simulink model "model"  (R2014a)
(part 7 of 8)

      | %<ID>
      | %<Vbase>V
      | %<VLF>pu
      | %<angleLF>deg.
      | %<Name>
  bus357 : powerlib/Measurements/Load Flow Bus  LConnTagsString=a  ID=bus357  Vbase=110000  Vref=1  Vangle=0  VLF=1  angleLF=0
      settings: AttributesFormatString=|
      | %<ID>
      | %<Vbase>V
      | %<VLF>pu
      | %<angleLF>deg.
      | %<Name>
  bus358 : powerlib/Measurements/Load Flow Bus  LConnTagsString=a  ID=bus358  Vbase=110000  Vref=1  Vangle=0  VLF=1  angleLF=0
      settings: AttributesFormatString=|
      | %<ID>
      | %<Vbase>V
      | %<VLF>pu
      | %<angleLF>deg.
      | %<Name>
  bus359 : powerlib/Measurements/Load Flow Bus  LConnTagsString=a  ID=bus359  Vbase=110000  Vref=1  Vangle=0  VLF=1  angleLF=0
      settings: AttributesFormatString=|
      | %<ID>
      | %<Vbase>V
      | %<VLF>pu
      | %<angleLF>deg.
      | %<Name>
  bus36 : powerlib/Measurements/Load Flow Bus  LConnTagsString=a  ID=bus36  Vbase=110000  Vref=1  Vangle=0  VLF=1  angleLF=0
      settings: AttributesFormatString=|
      | %<ID>
      | %<Vbase>V
      | %<VLF>pu
      | %<angleLF>deg.
      | %<Name>
  bus360 : powerlib/Measurements/Load Flow Bus  LConnTagsString=a  ID=bus360  Vbase=110000  Vref=1  Vangle=0  VLF=1  angleLF=0
      settings: AttributesFormatString=|
      | %<ID>
      | %<Vbase>V
      | %<VLF>pu
      | %<angleLF>deg.
      | %<Name>
  bus361 : powerlib/Measurements/Load Flow Bus  LConnTagsString=a  ID=bus361  Vbase=110000  Vref=1  Vangle=0  VLF=1  angleLF=0
      settings: AttributesFormatString=|
      | %<ID>
      | %<Vbase>V
      | %<VLF>pu
      | %<angleLF>deg.
      | %<Name>
  bus362 : powerlib/Measurements/Load Flow Bus  LConnTagsString=a  ID=bus362  Vbase=110000  Vref=1  Vangle=0  VLF=1  angleLF=0
      settings: AttributesFormatString=|
      | %<ID>
      | %<Vbase>V
      | %<VLF>pu
      | %<angleLF>deg.
      | %<Name>
  bus363 : powerlib/Measurements/Load Flow Bus  LConnTagsString=a  ID=bus363  Vbase=110000  Vref=1  Vangle=0  VLF=1  angleLF=0
      settings: AttributesFormatString=|
      | %<ID>
      | %<Vbase>V
      | %<VLF>pu
      | %<angleLF>deg.
      | %<Name>
  bus364 : powerlib/Measurements/Load Flow Bus  LConnTagsString=a  ID=bus364  Vbase=110000  Vref=1  Vangle=0  VLF=1  angleLF=0
      settings: AttributesFormatString=|
      | %<ID>
      | %<Vbase>V
      | %<VLF>pu
      | %<angleLF>deg.
      | %<Name>
  bus365 : powerlib/Measurements/Load Flow Bus  LConnTagsString=a  ID=bus365  Vbase=110000  Vref=1  Vangle=0  VLF=1  angleLF=0
      settings: AttributesFormatString=|
      | %<ID>
      | %<Vbase>V
      | %<VLF>pu
      | %<angleLF>deg.
      | %<Name>
  bus366 : powerlib/Measurements/Load Flow Bus  LConnTagsString=a  ID=bus366  Vbase=110000  Vref=1  Vangle=0  VLF=1  angleLF=0
      settings: AttributesFormatString=|
      | %<ID>
      | %<Vbase>V
      | %<VLF>pu
      | %<angleLF>deg.
      | %<Name>
  bus367 : powerlib/Measurements/Load Flow Bus  LConnTagsString=a  ID=bus367  Vbase=110000  Vref=1  Vangle=0  VLF=1  angleLF=0
      settings: AttributesFormatString=|
      | %<ID>
      | %<Vbase>V
      | %<VLF>pu
      | %<angleLF>deg.
      | %<Name>
  bus368 : powerlib/Measurements/Load Flow Bus  LConnTagsString=a  ID=bus368  Vbase=110000  Vref=1  Vangle=0  VLF=1  angleLF=0
      settings: AttributesFormatString=|
      | %<ID>
      | %<Vbase>V
      | %<VLF>pu
      | %<angleLF>deg.
      | %<Name>
  bus369 : powerlib/Measurements/Load Flow Bus  LConnTagsString=a  ID=bus369  Vbase=110000  Vref=1  Vangle=0  VLF=1  angleLF=0
      settings: AttributesFormatString=|
      | %<ID>
      | %<Vbase>V
      | %<VLF>pu
      | %<angleLF>deg.
      | %<Name>
  bus37 : powerlib/Measurements/Load Flow Bus  LConnTagsString=a  ID=bus37  Vbase=110000  Vref=1  Vangle=0  VLF=1  angleLF=0
      settings: AttributesFormatString=|
      | %<ID>
      | %<Vbase>V
      | %<VLF>pu
      | %<angleLF>deg.
      | %<Name>
  bus370 : powerlib/Measurements/Load Flow Bus  LConnTagsString=a  ID=bus370  Vbase=110000  Vref=1  Vangle=0  VLF=1  angleLF=0
      settings: AttributesFormatString=|
      | %<ID>
      | %<Vbase>V
      | %<VLF>pu
      | %<angleLF>deg.
      | %<Name>
  bus371 : powerlib/Measurements/Load Flow Bus  LConnTagsString=a  ID=bus371  Vbase=110000  Vref=1  Vangle=0  VLF=1  angleLF=0
      settings: AttributesFormatString=|
      | %<ID>
      | %<Vbase>V
      | %<VLF>pu
      | %<angleLF>deg.
      | %<Name>
  bus372 : powerlib/Measurements/Load Flow Bus  LConnTagsString=a  ID=bus372  Vbase=110000  Vref=1  Vangle=0  VLF=1  angleLF=0
      settings: AttributesFormatString=|
      | %<ID>
      | %<Vbase>V
      | %<VLF>pu
      | %<angleLF>deg.
      | %<Name>
  bus373 : powerlib/Measurements/Load Flow Bus  LConnTagsString=a  ID=bus373  Vbase=110000  Vref=1  Vangle=0  VLF=1  angleLF=0
      settings: AttributesFormatString=|
      | %<ID>
      | %<Vbase>V
      | %<VLF>pu
      | %<angleLF>deg.
      | %<Name>
  bus374 : powerlib/Measurements/Load Flow Bus  LConnTagsString=a  ID=bus374  Vbase=110000  Vref=1  Vangle=0  VLF=1  angleLF=0
      settings: AttributesFormatString=|
      | %<ID>
      | %<Vbase>V
      | %<VLF>pu
      | %<angleLF>deg.
      | %<Name>
  bus375 : powerlib/Measurements/Load Flow Bus  LConnTagsString=a  ID=bus375  Vbase=110000  Vref=1  Vangle=0  VLF=1  angleLF=0
      settings: AttributesFormatString=|
      | %<ID>
      | %<Vbase>V
      | %<VLF>pu
      | %<angleLF>deg.
      | %<Name>
  bus376 : powerlib/Measurements/Load Flow Bus  LConnTagsString=a  ID=bus376  Vbase=110000  Vref=1  Vangle=0  VLF=1  angleLF=0
      settings: AttributesFormatString=|
      | %<ID>
      | %<Vbase>V
      | %<VLF>pu
      | %<angleLF>deg.
      | %<Name>
  bus377 : powerlib/Measurements/Load Flow Bus  LConnTagsString=a  ID=bus377  Vbase=110000  Vref=1  Vangle=0  VLF=1  angleLF=0
      settings: AttributesFormatString=|
      | %<ID>
      | %<Vbase>V
      | %<VLF>pu
      | %<angleLF>deg.
      | %<Name>
  bus378 : powerlib/Measurements/Load Flow Bus  LConnTagsString=a  ID=bus378  Vbase=110000  Vref=1  Vangle=0  VLF=1  angleLF=0
      settings: AttributesFormatString=|
      | %<ID>
      | %<Vbase>V
      | %<VLF>pu
      | %<angleLF>deg.
      | %<Name>
  bus379 : powerlib/Measurements/Load Flow Bus  LConnTagsString=a  ID=bus379  Vbase=110000  Vref=1  Vangle=0  VLF=1  angleLF=0
      settings: AttributesFormatString=|
      | %<ID>
      | %<Vbase>V
      | %<VLF>pu
      | %<angleLF>deg.
      | %<Name>
  bus38 : powerlib/Measurements/Load Flow Bus  LConnTagsString=a  ID=bus38  Vbase=110000  Vref=1  Vangle=0  VLF=1  angleLF=0
      settings: AttributesFormatString=|
      | %<ID>
      | %<Vbase>V
      | %<VLF>pu
      | %<angleLF>deg.
      | %<Name>
  bus380 : powerlib/Measurements/Load Flow Bus  LConnTagsString=a  ID=bus380  Vbase=110000  Vref=1  Vangle=0  VLF=1  angleLF=0
      settings: AttributesFormatString=|
      | %<ID>
      | %<Vbase>V
      | %<VLF>pu
      | %<angleLF>deg.
      | %<Name>
  bus381 : powerlib/Measurements/Load Flow Bus  LConnTagsString=a  ID=bus381  Vbase=110000  Vref=1  Vangle=0  VLF=1  angleLF=0
      settings: AttributesFormatString=|
      | %<ID>
      | %<Vbase>V
      | %<VLF>pu
      | %<angleLF>deg.
      | %<Name>
  bus382 : powerlib/Measurements/Load Flow Bus  LConnTagsString=a  ID=bus382  Vbase=110000  Vref=1  Vangle=0  VLF=1  angleLF=0
      settings: AttributesFormatString=|
      | %<ID>
      | %<Vbase>V
      | %<VLF>pu
      | %<angleLF>deg.
      | %<Name>
  bus383 : powerlib/Measurements/Load Flow Bus  LConnTagsString=a  ID=bus383  Vbase=110000  Vref=1  Vangle=0  VLF=1  angleLF=0
      settings: AttributesFormatString=|
      | %<ID>
      | %<Vbase>V
      | %<VLF>pu
      | %<angleLF>deg.
      | %<Name>
  bus384 : powerlib/Measurements/Load Flow Bus  LConnTagsString=a  ID=bus384  Vbase=110000  Vref=1  Vangle=0  VLF=1  angleLF=0
      settings: AttributesFormatString=|
      | %<ID>
      | %<Vbase>V
      | %<VLF>pu
      | %<angleLF>deg.
      | %<Name>
  bus385 : powerlib/Measurements/Load Flow Bus  LConnTagsString=a  ID=bus385  Vbase=110000  Vref=1  Vangle=0  VLF=1  angleLF=0
      settings: AttributesFormatString=|
      | %<ID>
      | %<Vbase>V
      | %<VLF>pu
      | %<angleLF>deg.
      | %<Name>
  bus386 : powerlib/Measurements/Load Flow Bus  LConnTagsString=a  ID=bus386  Vbase=110000  Vref=1  Vangle=0  VLF=1  angleLF=0
      settings: AttributesFormatString=|
      | %<ID>
      | %<Vbase>V
      | %<VLF>pu
      | %<angleLF>deg.
      | %<Name>
  bus387 : powerlib/Measurements/Load Flow Bus  LConnTagsString=a  ID=bus387  Vbase=110000  Vref=1  Vangle=0  VLF=1  angleLF=0
      settings: AttributesFormatString=|
      | %<ID>
      | %<Vbase>V
      | %<VLF>pu
      | %<angleLF>deg.
      | %<Name>
  bus388 : powerlib/Measurements/Load Flow Bus  LConnTagsString=a  ID=bus388  Vbase=110000  Vref=1  Vangle=0  VLF=1  angleLF=0
      settings: AttributesFormatString=|
      | %<ID>
      | %<Vbase>V
      | %<VLF>pu
      | %<angleLF>deg.
      | %<Name>
  bus389 : powerlib/Measurements/Load Flow Bus  LConnTagsString=a  ID=bus389  Vbase=110000  Vref=1  Vangle=0  VLF=1  angleLF=0
      settings: AttributesFormatString=|
      | %<ID>
      | %<Vbase>V
      | %<VLF>pu
      | %<angleLF>deg.
      | %<Name>
  bus39 : powerlib/Measurements/Load Flow Bus  LConnTagsString=a  ID=bus39  Vbase=110000  Vref=1  Vangle=0  VLF=1  angleLF=0
      settings: AttributesFormatString=|
      | %<ID>
      | %<Vbase>V
      | %<VLF>pu
      | %<angleLF>deg.
      | %<Name>
  bus390 : powerlib/Measurements/Load Flow Bus  LConnTagsString=a  ID=bus390  Vbase=110000  Vref=1  Vangle=0  VLF=1  angleLF=0
      settings: AttributesFormatString=|
      | %<ID>
      | %<Vbase>V
      | %<VLF>pu
      | %<angleLF>deg.
      | %<Name>
  bus391 : powerlib/Measurements/Load Flow Bus  LConnTagsString=a  ID=bus391  Vbase=110000  Vref=1  Vangle=0  VLF=1  angleLF=0
      settings: AttributesFormatString=|
      | %<ID>
      | %<Vbase>V
      | %<VLF>pu
      | %<angleLF>deg.
      | %<Name>
  bus392 : powerlib/Measurements/Load Flow Bus  LConnTagsString=a  ID=bus392  Vbase=110000  Vref=1  Vangle=0  VLF=1  angleLF=0
      settings: AttributesFormatString=|
      | %<ID>
      | %<Vbase>V
      | %<VLF>pu
      | %<angleLF>deg.
      | %<Name>
  bus393 : powerlib/Measurements/Load Flow Bus  LConnTagsString=a  ID=bus393  Vbase=110000  Vref=1  Vangle=0  VLF=1  angleLF=0
      settings: AttributesFormatString=|
      | %<ID>
      | %<Vbase>V
      | %<VLF>pu
      | %<angleLF>deg.
      | %<Name>
  bus394 : powerlib/Measurements/Load Flow Bus  LConnTagsString=a  ID=bus394  Vbase=110000  Vref=1  Vangle=0  VLF=1  angleLF=0
      settings: AttributesFormatString=|
      | %<ID>
      | %<Vbase>V
      | %<VLF>pu
      | %<angleLF>deg.
      | %<Name>
  bus395 : powerlib/Measurements/Load Flow Bus  LConnTagsString=a  ID=bus395  Vbase=110000  Vref=1  Vangle=0  VLF=1  angleLF=0
      settings: AttributesFormatString=|
      | %<ID>
      | %<Vbase>V
      | %<VLF>pu
      | %<angleLF>deg.
      | %<Name>
  bus396 : powerlib/Measurements/Load Flow Bus  LConnTagsString=a  ID=bus396  Vbase=110000  Vref=1  Vangle=0  VLF=1  angleLF=0
      settings: AttributesFormatString=|
      | %<ID>
      | %<Vbase>V
      | %<VLF>pu
      | %<angleLF>deg.
      | %<Name>
  bus397 : powerlib/Measurements/Load Flow Bus  LConnTagsString=a  ID=bus397  Vbase=110000  Vref=1  Vangle=0  VLF=1  angleLF=0
      settings: AttributesFormatString=|
      | %<ID>
      | %<Vbase>V
      | %<VLF>pu
      | %<angleLF>deg.
      | %<Name>
  bus398 : powerlib/Measurements/Load Flow Bus  LConnTagsString=a  ID=bus398  Vbase=110000  Vref=1  Vangle=0  VLF=1  angleLF=0
      settings: AttributesFormatString=|
      | %<ID>
      | %<Vbase>V
      | %<VLF>pu
      | %<angleLF>deg.
      | %<Name>
  bus399 : powerlib/Measurements/Load Flow Bus  LConnTagsString=a  ID=bus399  Vbase=110000  Vref=1  Vangle=0  VLF=1  angleLF=0
      settings: AttributesFormatString=|
      | %<ID>
      | %<Vbase>V
      | %<VLF>pu
      | %<angleLF>deg.
      | %<Name>
  bus4 : powerlib/Measurements/Load Flow Bus  LConnTagsString=a  ID=bus4  Vbase=20000  Vref=1  Vangle=0  VLF=1  angleLF=0
      settings: AttributesFormatString=|
      | %<ID>
      | %<Vbase>V
      | %<VLF>pu
      | %<angleLF>deg.
      | %<Name>
  bus40 : powerlib/Measurements/Load Flow Bus  LConnTagsString=a  ID=bus40  Vbase=110000  Vref=1  Vangle=0  VLF=1  angleLF=0
      settings: AttributesFormatString=|
      | %<ID>
      | %<Vbase>V
      | %<VLF>pu
      | %<angleLF>deg.
      | %<Name>
  bus400 : powerlib/Measurements/Load Flow Bus  LConnTagsString=a  ID=bus400  Vbase=110000  Vref=1  Vangle=0  VLF=1  angleLF=0
      settings: AttributesFormatString=|
      | %<ID>
      | %<Vbase>V
      | %<VLF>pu
      | %<angleLF>deg.
      | %<Name>
  bus401 : powerlib/Measurements/Load Flow Bus  LConnTagsString=a  ID=bus401  Vbase=110000  Vref=1  Vangle=0  VLF=1  angleLF=0
      settings: AttributesFormatString=|
      | %<ID>
      | %<Vbase>V
      | %<VLF>pu
      | %<angleLF>deg.
      | %<Name>
  bus402 : powerlib/Measurements/Load Flow Bus  LConnTagsString=a  ID=bus402  Vbase=110000  Vref=1  Vangle=0  VLF=1  angleLF=0
      settings: AttributesFormatString=|
      | %<ID>
      | %<Vbase>V
      | %<VLF>pu
      | %<angleLF>deg.
      | %<Name>
  bus403 : powerlib/Measurements/Load Flow Bus  LConnTagsString=a  ID=bus403  Vbase=110000  Vref=1  Vangle=0  VLF=1  angleLF=0
      settings: AttributesFormatString=|
      | %<ID>
      | %<Vbase>V
      | %<VLF>pu
      | %<angleLF>deg.
      | %<Name>
  bus404 : powerlib/Measurements/Load Flow Bus  LConnTagsString=a  ID=bus404  Vbase=110000  Vref=1  Vangle=0  VLF=1  angleLF=0
      settings: AttributesFormatString=|
      | %<ID>
      | %<Vbase>V
      | %<VLF>pu
      | %<angleLF>deg.
      | %<Name>
  bus405 : powerlib/Measurements/Load Flow Bus  LConnTagsString=a  ID=bus405  Vbase=110000  Vref=1  Vangle=0  VLF=1  angleLF=0
      settings: AttributesFormatString=|
      | %<ID>
      | %<Vbase>V
      | %<VLF>pu
      | %<angleLF>deg.
      | %<Name>
  bus406 : powerlib/Measurements/Load Flow Bus  LConnTagsString=a  ID=bus406  Vbase=110000  Vref=1  Vangle=0  VLF=1  angleLF=0
      settings: AttributesFormatString=|
      | %<ID>
      | %<Vbase>V
      | %<VLF>pu
      | %<angleLF>deg.
      | %<Name>
  bus407 : powerlib/Measurements/Load Flow Bus  LConnTagsString=a  ID=bus407  Vbase=110000  Vref=1  Vangle=0  VLF=1  angleLF=0
      settings: AttributesFormatString=|
      | %<ID>
      | %<Vbase>V
      | %<VLF>pu
      | %<angleLF>deg.
      | %<Name>
  bus408 : powerlib/Measurements/Load Flow Bus  LConnTagsString=a  ID=bus408  Vbase=110000  Vref=1  Vangle=0  VLF=1  angleLF=0
      settings: AttributesFormatString=|
      | %<ID>
      | %<Vbase>V
      | %<VLF>pu
      | %<angleLF>deg.
      | %<Name>
  bus409 : powerlib/Measurements/Load Flow Bus  LConnTagsString=a  ID=bus409  Vbase=110000  Vref=1  Vangle=0  VLF=1  angleLF=0
      settings: AttributesFormatString=|
      | %<ID>
      | %<Vbase>V
      | %<VLF>pu
      | %<angleLF>deg.
      | %<Name>
  bus41 : powerlib/Measurements/Load Flow Bus  LConnTagsString=a  ID=bus41  Vbase=110000  Vref=1  Vangle=0  VLF=1  angleLF=0
      settings: AttributesFormatString=|
      | %<ID>
      | %<Vbase>V
      | %<VLF>pu
      | %<angleLF>deg.
      | %<Name>
  bus410 : powerlib/Measurements/Load Flow Bus  LConnTagsString=a  ID=bus410  Vbase=110000  Vref=1  Vangle=0  VLF=1  angleLF=0
      settings: AttributesFormatString=|
      | %<ID>
      | %<Vbase>V
      | %<VLF>pu
      | %<angleLF>deg.
      | %<Name>
  bus411 : powerlib/Measurements/Load Flow Bus  LConnTagsString=a  ID=bus411  Vbase=110000  Vref=1  Vangle=0  VLF=1  angleLF=0
      settings: AttributesFormatString=|
      | %<ID>
      | %<Vbase>V
      | %<VLF>pu
      | %<angleLF>deg.
      | %<Name>
  bus412 : powerlib/Measurements/Load Flow Bus  LConnTagsString=a  ID=bus412  Vbase=110000  Vref=1  Vangle=0  VLF=1  angleLF=0
      settings: AttributesFormatString=|
      | %<ID>
      | %<Vbase>V
      | %<VLF>pu
      | %<angleLF>deg.
      | %<Name>
  bus413 : powerlib/Measurements/Load Flow Bus  LConnTagsString=a  ID=bus413  Vbase=110000  Vref=1  Vangle=0  VLF=1  angleLF=0
      settings: AttributesFormatString=|
      | %<ID>
      | %<Vbase>V
      | %<VLF>pu
      | %<angleLF>deg.
      | %<Name>
  bus414 : powerlib/Measurements/Load Flow Bus  LConnTagsString=a  ID=bus414  Vbase=110000  Vref=1  Vangle=0  VLF=1  angleLF=0
      settings: AttributesFormatString=|
      | %<ID>
      | %<Vbase>V
      | %<VLF>pu
      | %<angleLF>deg.
      | %<Name>
  bus415 : powerlib/Measurements/Load Flow Bus  LConnTagsString=a  ID=bus415  Vbase=110000  Vref=1  Vangle=0  VLF=1  angleLF=0
      settings: AttributesFormatString=|
      | %<ID>
      | %<Vbase>V
      | %<VLF>pu
      | %<angleLF>deg.
      | %<Name>
  bus416 : powerlib/Measurements/Load Flow Bus  LConnTagsString=a  ID=bus416  Vbase=110000  Vref=1  Vangle=0  VLF=1  angleLF=0
      settings: AttributesFormatString=|
      | %<ID>
      | %<Vbase>V
      | %<VLF>pu
      | %<angleLF>deg.
      | %<Name>
  bus417 : powerlib/Measurements/Load Flow Bus  LConnTagsString=a  ID=bus417  Vbase=110000  Vref=1  Vangle=0  VLF=1  angleLF=0
      settings: AttributesFormatString=|
      | %<ID>
      | %<Vbase>V
      | %<VLF>pu
      | %<angleLF>deg.
      | %<Name>
  bus418 : powerlib/Measurements/Load Flow Bus  LConnTagsString=a  ID=bus418  Vbase=110000  Vref=1  Vangle=0  VLF=1  angleLF=0
      settings: AttributesFormatString=|
      | %<ID>
      | %<Vbase>V
      | %<VLF>pu
      | %<angleLF>deg.
      | %<Name>
  bus419 : powerlib/Measurements/Load Flow Bus  LConnTagsString=a  ID=bus419  Vbase=110000  Vref=1  Vangle=0  VLF=1  angleLF=0
      settings: AttributesFormatString=|
      | %<ID>
      | %<Vbase>V
      | %<VLF>pu
      | %<angleLF>deg.
      | %<Name>
  bus42 : powerlib/Measurements/Load Flow Bus  LConnTagsString=a  ID=bus42  Vbase=110000  Vref=1  Vangle=0  VLF=1  angleLF=0
      settings: AttributesFormatString=|
      | %<ID>
      | %<Vbase>V
      | %<VLF>pu
      | %<angleLF>deg.
      | %<Name>
  bus420 : powerlib/Measurements/Load Flow Bus  LConnTagsString=a  ID=bus420  Vbase=110000  Vref=1  Vangle=0  VLF=1  angleLF=0
      settings: AttributesFormatString=|
      | %<ID>
      | %<Vbase>V
      | %<VLF>pu
      | %<angleLF>deg.
      | %<Name>
  bus421 : powerlib/Measurements/Load Flow Bus  LConnTagsString=a  ID=bus421  Vbase=110000  Vref=1  Vangle=0  VLF=1  angleLF=0
      settings: AttributesFormatString=|
      | %<ID>
      | %<Vbase>V
      | %<VLF>pu
      | %<angleLF>deg.
      | %<Name>
  bus422 : powerlib/Measurements/Load Flow Bus  LConnTagsString=a  ID=bus422  Vbase=110000  Vref=1  Vangle=0  VLF=1  angleLF=0
      settings: AttributesFormatString=|
      | %<ID>
      | %<Vbase>V
      | %<VLF>pu
      | %<angleLF>deg.
      | %<Name>
  bus423 : powerlib/Measurements/Load Flow Bus  LConnTagsString=a  ID=bus423  Vbase=110000  Vref=1  Vangle=0  VLF=1  angleLF=0
      settings: AttributesFormatString=|
      | %<ID>
      | %<Vbase>V
      | %<VLF>pu
      | %<angleLF>deg.
      | %<Name>
  bus424 : powerlib/Measurements/Load Flow Bus  LConnTagsString=a  ID=bus424  Vbase=110000  Vref=1  Vangle=0  VLF=1  angleLF=0
      settings: AttributesFormatString=|
      | %<ID>
      | %<Vbase>V
      | %<VLF>pu
      | %<angleLF>deg.
      | %<Name>
  bus425 : powerlib/Measurements/Load Flow Bus  LConnTagsString=a  ID=bus425  Vbase=110000  Vref=1  Vangle=0  VLF=1  angleLF=0
      settings: AttributesFormatString=|
      | %<ID>
      | %<Vbase>V
      | %<VLF>pu
      | %<angleLF>deg.
      | %<Name>
  bus426 : powerlib/Measurements/Load Flow Bus  LConnTagsString=a  ID=bus426  Vbase=110000  Vref=1  Vangle=0  VLF=1  angleLF=0
      settings: AttributesFormatString=|
      | %<ID>
      | %<Vbase>V
      | %<VLF>pu
      | %<angleLF>deg.
      | %<Name>
  bus427 : powerlib/Measurements/Load Flow Bus  LConnTagsString=a  ID=bus427  Vbase=110000  Vref=1  Vangle=0  VLF=1  angleLF=0
      settings: AttributesFormatString=|
      | %<ID>
      | %<Vbase>V
      | %<VLF>pu
      | %<angleLF>deg.
      | %<Name>
  bus428 : powerlib/Measurements/Load Flow Bus  LConnTagsString=a  ID=bus428  Vbase=110000  Vref=1  Vangle=0  VLF=1  angleLF=0
      settings: AttributesFormatString=|
      | %<ID>
      | %<Vbase>V
      | %<VLF>pu
      | %<angleLF>deg.
      | %<Name>
  bus429 : powerlib/Measurements/Load Flow Bus  LConnTagsString=a  ID=bus429  Vbase=110000  Vref=1  Vangle=0  VLF=1  angleLF=0
      settings: AttributesFormatString=|
      | %<ID>
      | %<Vbase>V
      | %<VLF>pu
      | %<angleLF>deg.
      | %<Name>
  bus43 : powerlib/Measurements/Load Flow Bus  LConnTagsString=a  ID=bus43  Vbase=110000  Vref=1  Vangle=0  VLF=1  angleLF=0
      settings: AttributesFormatString=|
      | %<ID>
      | %<Vbase>V
      | %<VLF>pu
      | %<angleLF>deg.
      | %<Name>
  bus430 : powerlib/Measurements/Load Flow Bus  LConnTagsString=a  ID=bus430  Vbase=110000  Vref=1  Vangle=0  VLF=1  angleLF=0
      settings: AttributesFormatString=|
      | %<ID>
      | %<Vbase>V
      | %<VLF>pu
      | %<angleLF>deg.
      | %<Name>
  bus431 : powerlib/Measurements/Load Flow Bus  LConnTagsString=a  ID=bus431  Vbase=110000  Vref=1  Vangle=0  VLF=1  angleLF=0
      settings: AttributesFormatString=|
      | %<ID>
      | %<Vbase>V
      | %<VLF>pu
      | %<angleLF>deg.
      | %<Name>
  bus432 : powerlib/Measurements/Load Flow Bus  LConnTagsString=a  ID=bus432  Vbase=110000  Vref=1  Vangle=0  VLF=1  angleLF=0
      settings: AttributesFormatString=|
      | %<ID>
      | %<Vbase>V
      | %<VLF>pu
      | %<angleLF>deg.
      | %<Name>
  bus433 : powerlib/Measurements/Load Flow Bus  LConnTagsString=a  ID=bus433  Vbase=110000  Vref=1  Vangle=0  VLF=1  angleLF=0
      settings: AttributesFormatString=|
      | %<ID>
      | %<Vbase>V
      | %<VLF>pu
      | %<angleLF>deg.
      | %<Name>
  bus434 : powerlib/Measurements/Load Flow Bus  LConnTagsString=a  ID=bus434  Vbase=110000  Vref=1  Vangle=0  VLF=1  angleLF=0
      settings: AttributesFormatString=|
      | %<ID>
      | %<Vbase>V
      | %<VLF>pu
      | %<angleLF>deg.
      | %<Name>
  bus435 : powerlib/Measurements/Load Flow Bus  LConnTagsString=a  ID=bus435  Vbase=110000  Vref=1  Vangle=0  VLF=1  angleLF=0
      settings: AttributesFormatString=|
      | %<ID>
      | %<Vbase>V
      | %<VLF>pu
      | %<angleLF>deg.
      | %<Name>
  bus436 : powerlib/Measurements/Load Flow Bus  LConnTagsString=a  ID=bus436  Vbase=110000  Vref=1  Vangle=0  VLF=1  angleLF=0
      settings: AttributesFormatString=|
      | %<ID>
      | %<Vbase>V
      | %<VLF>pu
      | %<angleLF>deg.
      | %<Name>
  bus437 : powerlib/Measurements/Load Flow Bus  LConnTagsString=a  ID=bus437  Vbase=110000  Vref=1  Vangle=0  VLF=1  angleLF=0
      settings: AttributesFormatString=|
      | %<ID>
      | %<Vbase>V
      | %<VLF>pu
      | %<angleLF>deg.
      | %<Name>
  bus438 : powerlib/Measurements/Load Flow Bus  LConnTagsString=a  ID=bus438  Vbase=110000  Vref=1  Vangle=0  VLF=1  angleLF=0
      settings: AttributesFormatString=|
      | %<ID>
      | %<Vbase>V
      | %<VLF>pu
      | %<angleLF>deg.
      | %<Name>
  bus439 : powerlib/Measurements/Load Flow Bus  LConnTagsString=a  ID=bus439  Vbase=110000  Vref=1  Vangle=0  VLF=1  angleLF=0
      settings: AttributesFormatString=|
      | %<ID>
      | %<Vbase>V
      | %<VLF>pu
      | %<angleLF>deg.
      | %<Name>
  bus44 : powerlib/Measurements/Load Flow Bus  LConnTagsString=a  ID=bus44  Vbase=110000  Vref=1  Vangle=0  VLF=1  angleLF=0
      settings: AttributesFormatString=|
      | %<ID>
      | %<Vbase>V
      | %<VLF>pu
      | %<angleLF>deg.
      | %<Name>
  bus440 : powerlib/Measurements/Load Flow Bus  LConnTagsString=a  ID=bus440  Vbase=110000  Vref=1  Vangle=0  VLF=1  angleLF=0
      settings: AttributesFormatString=|
      | %<ID>
      | %<Vbase>V
      | %<VLF>pu
      | %<angleLF>deg.
      | %<Name>
  bus441 : powerlib/Measurements/Load Flow Bus  LConnTagsString=a  ID=bus441  Vbase=110000  Vref=1  Vangle=0  VLF=1  angleLF=0
      settings: AttributesFormatString=|
      | %<ID>
      | %<Vbase>V
      | %<VLF>pu
      | %<angleLF>deg.
      | %<Name>
  bus442 : powerlib/Measurements/Load Flow Bus  LConnTagsString=a  ID=bus442  Vbase=110000  Vref=1  Vangle=0  VLF=1  angleLF=0
      settings: AttributesFormatString=|
      | %<ID>
      | %<Vbase>V
      | %<VLF>pu
      | %<angleLF>deg.
      | %<Name>
  bus443 : powerlib/Measurements/Load Flow Bus  LConnTagsString=a  ID=bus443  Vbase=110000  Vref=1  Vangle=0  VLF=1  angleLF=0
      settings: AttributesFormatString=|
      | %<ID>
      | %<Vbase>V
      | %<VLF>pu
      | %<angleLF>deg.
      | %<Name>
  bus444 : powerlib/Measurements/Load Flow Bus  LConnTagsString=a  ID=bus444  Vbase=110000  Vref=1  Vangle=0  VLF=1  angleLF=0
      settings: AttributesFormatString=|
      | %<ID>
      | %<Vbase>V
      | %<VLF>pu
      | %<angleLF>deg.
      | %<Name>
  bus445 : powerlib/Measurements/Load Flow Bus  LConnTagsString=a  ID=bus445  Vbase=110000  Vref=1  Vangle=0  VLF=1  angleLF=0
      settings: AttributesFormatString=|
      | %<ID>
      | %<Vbase>V
      | %<VLF>pu
      | %<angleLF>deg.
      | %<Name>
  bus446 : powerlib/Measurements/Load Flow Bus  LConnTagsString=a  ID=bus446  Vbase=110000  Vref=1  Vangle=0  VLF=1  angleLF=0
      settings: AttributesFormatString=|
      | %<ID>
      | %<Vbase>V
      | %<VLF>pu
      | %<angleLF>deg.
      | %<Name>
  bus447 : powerlib/Measurements/Load Flow Bus  LConnTagsString=a  ID=bus447  Vbase=110000  Vref=1  Vangle=0  VLF=1  angleLF=0
      settings: AttributesFormatString=|
      | %<ID>
      | %<Vbase>V
      | %<VLF>pu
      | %<angleLF>deg.
      | %<Name>
  bus448 : powerlib/Measurements/Load Flow Bus  LConnTagsString=a  ID=bus448  Vbase=110000  Vref=1  Vangle=0  VLF=1  angleLF=0
      settings: AttributesFormatString=|
      | %<ID>
      | %<Vbase>V
      | %<VLF>pu
      | %<angleLF>deg.
      | %<Name>
  bus449 : powerlib/Measurements/Load Flow Bus  LConnTagsString=a  ID=bus449  Vbase=110000  Vref=1  Vangle=0  VLF=1  angleLF=0
      settings: AttributesFormatString=|
      | %<ID>
      | %<Vbase>V
      | %<VLF>pu
      | %<angleLF>deg.
      | %<Name>
  bus45 : powerlib/Measurements/Load Flow Bus  LConnTagsString=a  ID=bus45  Vbase=110000  Vref=1  Vangle=0  VLF=1  angleLF=0
      settings: AttributesFormatString=|
      | %<ID>
      | %<Vbase>V
      | %<VLF>pu
      | %<angleLF>deg.
      | %<Name>
  bus450 : powerlib/Measurements/Load Flow Bus  LConnTagsString=a  ID=bus450  Vbase=110000  Vref=1  Vangle=0  VLF=1  angleLF=0
      settings: AttributesFormatString=|
      | %<ID>
      | %<Vbase>V
      | %<VLF>pu
      | %<angleLF>deg.
      | %<Name>
  bus451 : powerlib/Measurements/Load Flow Bus  LConnTagsString=a  ID=bus451  Vbase=110000  Vref=1  Vangle=0  VLF=1  angleLF=0
      settings: AttributesFormatString=|
      | %<ID>
      | %<Vbase>V
      | %<VLF>pu
      | %<angleLF>deg.
      | %<Name>
  bus452 : powerlib/Measurements/Load Flow Bus  LConnTagsString=a  ID=bus452  Vbase=110000  Vref=1  Vangle=0  VLF=1  angleLF=0
      settings: AttributesFormatString=|
      | %<ID>
      | %<Vbase>V
      | %<VLF>pu
      | %<angleLF>deg.
      | %<Name>
  bus453 : powerlib/Measurements/Load Flow Bus  LConnTagsString=a  ID=bus453  Vbase=110000  Vref=1  Vangle=0  VLF=1  angleLF=0
      settings: AttributesFormatString=|
      | %<ID>
      | %<Vbase>V
      | %<VLF>pu
      | %<angleLF>deg.
      | %<Name>
  bus454 : powerlib/Measurements/Load Flow Bus  LConnTagsString=a  ID=bus454  Vbase=110000  Vref=1  Vangle=0  VLF=1  angleLF=0
      settings: AttributesFormatString=|
      | %<ID>
      | %<Vbase>V
      | %<VLF>pu
      | %<angleLF>deg.
      | %<Name>
  bus455 : powerlib/Measurements/Load Flow Bus  LConnTagsString=a  ID=bus455  Vbase=110000  Vref=1  Vangle=0  VLF=1  angleLF=0
      settings: AttributesFormatString=|
      | %<ID>
      | %<Vbase>V
      | %<VLF>pu
      | %<angleLF>deg.
      | %<Name>
  bus456 : powerlib/Measurements/Load Flow Bus  LConnTagsString=a  ID=bus456  Vbase=110000  Vref=1  Vangle=0  VLF=1  angleLF=0
      settings: AttributesFormatString=|
      | %<ID>
      | %<Vbase>V
      | %<VLF>pu
      | %<angleLF>deg.
      | %<Name>
  bus457 : powerlib/Measurements/Load Flow Bus  LConnTagsString=a  ID=bus457  Vbase=110000  Vref=1  Vangle=0  VLF=1  angleLF=0
      settings: AttributesFormatString=|
      | %<ID>
      | %<Vbase>V
      | %<VLF>pu
      | %<angleLF>deg.
      | %<Name>
  bus458 : powerlib/Measurements/Load Flow Bus  LConnTagsString=a  ID=bus458  Vbase=110000  Vref=1  Vangle=0  VLF=1  angleLF=0
      settings: AttributesFormatString=|
      | %<ID>
      | %<Vbase>V
      | %<VLF>pu
      | %<angleLF>deg.
      | %<Name>
  bus459 : powerlib/Measurements/Load Flow Bus  LConnTagsString=a  ID=bus459  Vbase=110000  Vref=1  Vangle=0  VLF=1  angleLF=0
      settings: AttributesFormatString=|
      | %<ID>
      | %<Vbase>V
      | %<VLF>pu
      | %<angleLF>deg.
      | %<Name>
  bus46 : powerlib/Measurements/Load Flow Bus  LConnTagsString=a  ID=bus46  Vbase=110000  Vref=1  Vangle=0  VLF=1  angleLF=0
      settings: AttributesFormatString=|
      | %<ID>
      | %<Vbase>V
      | %<VLF>pu
      | %<angleLF>deg.
      | %<Name>
  bus460 : powerlib/Measurements/Load Flow Bus  LConnTagsString=a  ID=bus460  Vbase=110000  Vref=1  Vangle=0  VLF=1  angleLF=0
      settings: AttributesFormatString=|
      | %<ID>
      | %<Vbase>V
      | %<VLF>pu
      | %<angleLF>deg.
      | %<Name>
  bus461 : powerlib/Measurements/Load Flow Bus  LConnTagsString=a  ID=bus461  Vbase=110000  Vref=1  Vangle=0  VLF=1  angleLF=0
      settings: AttributesFormatString=|
      | %<ID>
      | %<Vbase>V
      | %<VLF>pu
      | %<angleLF>deg.
      | %<Name>
  bus462 : powerlib/Measurements/Load Flow Bus  LConnTagsString=a  ID=bus462  Vbase=110000  Vref=1  Vangle=0  VLF=1  angleLF=0
      settings: AttributesFormatString=|
      | %<ID>
      | %<Vbase>V
      | %<VLF>pu
      | %<angleLF>deg.
      | %<Name>
  bus463 : powerlib/Measurements/Load Flow Bus  LConnTagsString=a  ID=bus463  Vbase=110000  Vref=1  Vangle=0  VLF=1  angleLF=0
      settings: AttributesFormatString=|
      | %<ID>
      | %<Vbase>V
      | %<VLF>pu
      | %<angleLF>deg.
      | %<Name>
  bus464 : powerlib/Measurements/Load Flow Bus  LConnTagsString=a  ID=bus464  Vbase=110000  Vref=1  Vangle=0  VLF=1  angleLF=0
      settings: AttributesFormatString=|
      | %<ID>
      | %<Vbase>V
      | %<VLF>pu
      | %<angleLF>deg.
      | %<Name>
  bus465 : powerlib/Measurements/Load Flow Bus  LConnTagsString=a  ID=bus465  Vbase=110000  Vref=1  Vangle=0  VLF=1  angleLF=0
      settings: AttributesFormatString=|
      | %<ID>
      | %<Vbase>V
      | %<VLF>pu
      | %<angleLF>deg.
      | %<Name>
  bus466 : powerlib/Measurements/Load Flow Bus  LConnTagsString=a  ID=bus466  Vbase=110000  Vref=1  Vangle=0  VLF=1  angleLF=0
      settings: AttributesFormatString=|
      | %<ID>
      | %<Vbase>V
      | %<VLF>pu
      | %<angleLF>deg.
      | %<Name>
  bus467 : powerlib/Measurements/Load Flow Bus  LConnTagsString=a  ID=bus467  Vbase=110000  Vref=1  Vangle=0  VLF=1  angleLF=0
      settings: AttributesFormatString=|
      | %<ID>
      | %<Vbase>V
      | %<VLF>pu
      | %<angleLF>deg.
      | %<Name>
  bus468 : powerlib/Measurements/Load Flow Bus  LConnTagsString=a  ID=bus468  Vbase=110000  Vref=1  Vangle=0  VLF=1  angleLF=0
      settings: AttributesFormatString=|
      | %<ID>
      | %<Vbase>V
      | %<VLF>pu
      | %<angleLF>deg.
      | %<Name>
  bus469 : powerlib/Measurements/Load Flow Bus  LConnTagsString=a  ID=bus469  Vbase=110000  Vref=1  Vangle=0  VLF=1  angleLF=0
      settings: AttributesFormatString=|
      | %<ID>
      | %<Vbase>V
      | %<VLF>pu
      | %<angleLF>deg.
      | %<Name>
  bus47 : powerlib/Measurements/Load Flow Bus  LConnTagsString=a  ID=bus47  Vbase=110000  Vref=1  Vangle=0  VLF=1  angleLF=0
      settings: AttributesFormatString=|
      | %<ID>
      | %<Vbase>V
      | %<VLF>pu
      | %<angleLF>deg.
      | %<Name>
  bus470 : powerlib/Measurements/Load Flow Bus  LConnTagsString=a  ID=bus470  Vbase=110000  Vref=1  Vangle=0  VLF=1  angleLF=0
      settings: AttributesFormatString=|
      | %<ID>
      | %<Vbase>V
      | %<VLF>pu
      | %<angleLF>deg.
      | %<Name>
  bus471 : powerlib/Measurements/Load Flow Bus  LConnTagsString=a  ID=bus471  Vbase=110000  Vref=1  Vangle=0  VLF=1  angleLF=0
      settings: AttributesFormatString=|
      | %<ID>
      | %<Vbase>V
      | %<VLF>pu
      | %<angleLF>deg.
      | %<Name>
  bus472 : powerlib/Measurements/Load Flow Bus  LConnTagsString=a  ID=bus472  Vbase=110000  Vref=1  Vangle=0  VLF=1  angleLF=0
      settings: AttributesFormatString=|
      | %<ID>
      | %<Vbase>V
      | %<VLF>pu
      | %<angleLF>deg.
      | %<Name>
  bus473 : powerlib/Measurements/Load Flow Bus  LConnTagsString=a  ID=bus473  Vbase=110000  Vref=1  Vangle=0  VLF=1  angleLF=0
      settings: AttributesFormatString=|
      | %<ID>
      | %<Vbase>V
      | %<VLF>pu
      | %<angleLF>deg.
      | %<Name>
  bus474 : powerlib/Measurements/Load Flow Bus  LConnTagsString=a  ID=bus474  Vbase=110000  Vref=1  Vangle=0  VLF=1  angleLF=0
      settings: AttributesFormatString=|
      | %<ID>
      | %<Vbase>V
      | %<VLF>pu
      | %<angleLF>deg.
      | %<Name>
  bus475 : powerlib/Measurements/Load Flow Bus  LConnTagsString=a  ID=bus475  Vbase=110000  Vref=1  Vangle=0  VLF=1  angleLF=0
      settings: AttributesFormatString=|
      | %<ID>
      | %<Vbase>V
      | %<VLF>pu
      | %<angleLF>deg.
      | %<Name>
  bus476 : powerlib/Measurements/Load Flow Bus  LConnTagsString=a  ID=bus476  Vbase=110000  Vref=1  Vangle=0  VLF=1  angleLF=0
      settings: AttributesFormatString=|
      | %<ID>
      | %<Vbase>V
      | %<VLF>pu
      | %<angleLF>deg.
      | %<Name>
  bus477 : powerlib/Measurements/Load Flow Bus  LConnTagsString=a  ID=bus477  Vbase=110000  Vref=1  Vangle=0  VLF=1  angleLF=0
      settings: AttributesFormatString=|
      | %<ID>
      | %<Vbase>V
      | %<VLF>pu
      | %<angleLF>deg.
      | %<Name>
  bus478 : powerlib/Measurements/Load Flow Bus  LConnTagsString=a  ID=bus478  Vbase=110000  Vref=1  Vangle=0  VLF=1  angleLF=0
      settings: AttributesFormatString=|
      | %<ID>
      | %<Vbase>V
      | %<VLF>pu
      | %<angleLF>deg.
      | %<Name>
  bus479 : powerlib/Measurements/Load Flow Bus  LConnTagsString=a  ID=bus479  Vbase=110000  Vref=1  Vangle=0  VLF=1  angleLF=0
      settings: AttributesFormatString=|
      | %<ID>
      | %<Vbase>V
      | %<VLF>pu
      | %<angleLF>deg.
      | %<Name>
  bus48 : powerlib/Measurements/Load Flow Bus  LConnTagsString=a  ID=bus48  Vbase=110000  Vref=1  Vangle=0  VLF=1  angleLF=0
      settings: AttributesFormatString=|
      | %<ID>
      | %<Vbase>V
      | %<VLF>pu
      | %<angleLF>deg.
      | %<Name>
  bus480 : powerlib/Measurements/Load Flow Bus  LConnTagsString=a  ID=bus480  Vbase=110000  Vref=1  Vangle=0  VLF=1  angleLF=0
      settings: AttributesFormatString=|
      | %<ID>
      | %<Vbase>V
      | %<VLF>pu
      | %<angleLF>deg.
      | %<Name>
  bus481 : powerlib/Measurements/Load Flow Bus  LConnTagsString=a  ID=bus481  Vbase=110000  Vref=1  Vangle=0  VLF=1  angleLF=0
      settings: AttributesFormatString=|
      | %<ID>
      | %<Vbase>V
      | %<VLF>pu
      | %<angleLF>deg.
      | %<Name>
  bus482 : powerlib/Measurements/Load Flow Bus  LConnTagsString=a  ID=bus482  Vbase=110000  Vref=1  Vangle=0  VLF=1  angleLF=0
      settings: AttributesFormatString=|
      | %<ID>
      | %<Vbase>V
      | %<VLF>pu
      | %<angleLF>deg.
      | %<Name>
  bus483 : powerlib/Measurements/Load Flow Bus  LConnTagsString=a  ID=bus483  Vbase=110000  Vref=1  Vangle=0  VLF=1  angleLF=0
      settings: AttributesFormatString=|
      | %<ID>
      | %<Vbase>V
      | %<VLF>pu
      | %<angleLF>deg.
      | %<Name>
  bus484 : powerlib/Measurements/Load Flow Bus  LConnTagsString=a  ID=bus484  Vbase=110000  Vref=1  Vangle=0  VLF=1  angleLF=0
      settings: AttributesFormatString=|
      | %<ID>
      | %<Vbase>V
      | %<VLF>pu
      | %<angleLF>deg.
      | %<Name>
  bus485 : powerlib/Measurements/Load Flow Bus  LConnTagsString=a  ID=bus485  Vbase=110000  Vref=1  Vangle=0  VLF=1  angleLF=0
      settings: AttributesFormatString=|
      | %<ID>
      | %<Vbase>V
      | %<VLF>pu
      | %<angleLF>deg.
      | %<Name>
  bus486 : powerlib/Measurements/Load Flow Bus  LConnTagsString=a  ID=bus486  Vbase=110000  Vref=1  Vangle=0  VLF=1  angleLF=0
      settings: AttributesFormatString=|
      | %<ID>
      | %<Vbase>V
      | %<VLF>pu
      | %<angleLF>deg.
      | %<Name>
  bus487 : powerlib/Measurements/Load Flow Bus  LConnTagsString=a  ID=bus487  Vbase=110000  Vref=1  Vangle=0  VLF=1  angleLF=0
      settings: AttributesFormatString=|
      | %<ID>
      | %<Vbase>V
      | %<VLF>pu
      | %<angleLF>deg.
      | %<Name>
  bus488 : powerlib/Measurements/Load Flow Bus  LConnTagsString=a  ID=bus488  Vbase=110000  Vref=1  Vangle=0  VLF=1  angleLF=0
      settings: AttributesFormatString=|
      | %<ID>
      | %<Vbase>V
      | %<VLF>pu
      | %<angleLF>deg.
      | %<Name>
  bus489 : powerlib/Measurements/Load Flow Bus  LConnTagsString=a  ID=bus489  Vbase=110000  Vref=1  Vangle=0  VLF=1  angleLF=0
      settings: AttributesFormatString=|
      | %<ID>
      | %<Vbase>V
      | %<VLF>pu
      | %<angleLF>deg.
      | %<Name>
  bus49 : powerlib/Measurements/Load Flow Bus  LConnTagsString=a  ID=bus49  Vbase=110000  Vref=1  Vangle=0  VLF=1  angleLF=0
      settings: AttributesFormatString=|
      | %<ID>
      | %<Vbase>V
      | %<VLF>pu
      | %<angleLF>deg.
      | %<Name>
  bus490 : powerlib/Measurements/Load Flow Bus  LConnTagsString=a  ID=bus490  Vbase=110000  Vref=1  Vangle=0  VLF=1  angleLF=0
      settings: AttributesFormatString=|
      | %<ID>
      | %<Vbase>V
      | %<VLF>pu
      | %<angleLF>deg.
      | %<Name>
  bus491 : powerlib/Measurements/Load Flow Bus  LConnTagsString=a  ID=bus491  Vbase=110000  Vref=1  Vangle=0  VLF=1  angleLF=0
      settings: AttributesFormatString=|
      | %<ID>
      | %<Vbase>V
      | %<VLF>pu
      | %<angleLF>deg.
      | %<Name>
  bus492 : powerlib/Measurements/Load Flow Bus  LConnTagsString=a  ID=bus492  Vbase=110000  Vref=1  Vangle=0  VLF=1  angleLF=0
      settings: AttributesFormatString=|
      | %<ID>
      | %<Vbase>V
      | %<VLF>pu
      | %<angleLF>deg.
      | %<Name>
  bus493 : powerlib/Measurements/Load Flow Bus  LConnTagsString=a  ID=bus493  Vbase=110000  Vref=1  Vangle=0  VLF=1  angleLF=0
      settings: AttributesFormatString=|
      | %<ID>
      | %<Vbase>V
      | %<VLF>pu
      | %<angleLF>deg.
      | %<Name>
  bus494 : powerlib/Measurements/Load Flow Bus  LConnTagsString=a  ID=bus494  Vbase=110000  Vref=1  Vangle=0  VLF=1  angleLF=0
      settings: AttributesFormatString=|
      | %<ID>
      | %<Vbase>V
      | %<VLF>pu
      | %<angleLF>deg.
      | %<Name>
  bus495 : powerlib/Measurements/Load Flow Bus  LConnTagsString=a  ID=bus495  Vbase=110000  Vref=1  Vangle=0  VLF=1  angleLF=0
      settings: AttributesFormatString=|
      | %<ID>
      | %<Vbase>V
      | %<VLF>pu
      | %<angleLF>deg.
      | %<Name>
  bus496 : powerlib/Measurements/Load Flow Bus  LConnTagsString=a  ID=bus496  Vbase=110000  Vref=1  Vangle=0  VLF=1  angleLF=0
      settings: AttributesFormatString=|
      | %<ID>
      | %<Vbase>V
      | %<VLF>pu
      | %<angleLF>deg.
      | %<Name>
  bus497 : powerlib/Measurements/Load Flow Bus  LConnTagsString=a  ID=bus497  Vbase=110000  Vref=1  Vangle=0  VLF=1  angleLF=0
      settings: AttributesFormatString=|
      | %<ID>
      | %<Vbase>V
      | %<VLF>pu
      | %<angleLF>deg.
      | %<Name>
  bus498 : powerlib/Measurements/Load Flow Bus  LConnTagsString=a  ID=bus498  Vbase=110000  Vref=1  Vangle=0  VLF=1  angleLF=0
      settings: AttributesFormatString=|
      | %<ID>
      | %<Vbase>V
      | %<VLF>pu
      | %<angleLF>deg.
      | %<Name>
  bus499 : powerlib/Measurements/Load Flow Bus  LConnTagsString=a  ID=bus499  Vbase=110000  Vref=1  Vangle=0  VLF=1  angleLF=0
      settings: AttributesFormatString=|
      | %<ID>
      | %<Vbase>V
      | %<VLF>pu
      | %<angleLF>deg.
      | %<Name>
  bus5 : powerlib/Measurements/Load Flow Bus  LConnTagsString=a  ID=bus5  Vbase=20000  Vref=1  Vangle=0  VLF=1  angleLF=0
      settings: AttributesFormatString=|
      | %<ID>
      | %<Vbase>V
      | %<VLF>pu
      | %<angleLF>deg.
      | %<Name>
  bus50 : powerlib/Measurements/Load Flow Bus  LConnTagsString=a  ID=bus50  Vbase=110000  Vref=1  Vangle=0  VLF=1  angleLF=0
      settings: AttributesFormatString=|
      | %<ID>
      | %<Vbase>V
      | %<VLF>pu
      | %<angleLF>deg.
      | %<Name>
  bus500 : powerlib/Measurements/Load Flow Bus  LConnTagsString=a  ID=bus500  Vbase=110000  Vref=1  Vangle=0  VLF=1  angleLF=0
      settings: AttributesFormatString=|
      | %<ID>
      | %<Vbase>V
      | %<VLF>pu
      | %<angleLF>deg.
      | %<Name>
  bus501 : powerlib/Measurements/Load Flow Bus  LConnTagsString=a  ID=bus501  Vbase=110000  Vref=1  Vangle=0  VLF=1  angleLF=0
      settings: AttributesFormatString=|
      | %<ID>
      | %<Vbase>V
      | %<VLF>pu
      | %<angleLF>deg.
      | %<Name>
  bus502 : powerlib/Measurements/Load Flow Bus  LConnTagsString=a  ID=bus502  Vbase=110000  Vref=1  Vangle=0  VLF=1  angleLF=0
      settings: AttributesFormatString=|
      | %<ID>
      | %<Vbase>V
      | %<VLF>pu
      | %<angleLF>deg.
      | %<Name>
  bus503 : powerlib/Measurements/Load Flow Bus  LConnTagsString=a  ID=bus503  Vbase=110000  Vref=1  Vangle=0  VLF=1  angleLF=0
      settings: AttributesFormatString=|
      | %<ID>
      | %<Vbase>V
      | %<VLF>pu
      | %<angleLF>deg.
      | %<Name>
  bus504 : powerlib/Measurements/Load Flow Bus  LConnTagsString=a  ID=bus504  Vbase=110000  Vref=1  Vangle=0  VLF=1  angleLF=0
      settings: AttributesFormatString=|
      | %<ID>
      | %<Vbase>V
      | %<VLF>pu
      | %<angleLF>deg.
      | %<Name>
  bus505 : powerlib/Measurements/Load Flow Bus  LConnTagsString=a  ID=bus505  Vbase=110000  Vref=1  Vangle=0  VLF=1  angleLF=0
      settings: AttributesFormatString=|
      | %<ID>
      | %<Vbase>V
      | %<VLF>pu
      | %<angleLF>deg.
      | %<Name>
  bus506 : powerlib/Measurements/Load Flow Bus  LConnTagsString=a  ID=bus506  Vbase=110000  Vref=1  Vangle=0  VLF=1  angleLF=0
      settings: AttributesFormatString=|
      | %<ID>
      | %<Vbase>V
      | %<VLF>pu
      | %<angleLF>deg.
      | %<Name>
  bus507 : powerlib/Measurements/Load Flow Bus  LConnTagsString=a  ID=bus507  Vbase=110000  Vref=1  Vangle=0  VLF=1  angleLF=0
      settings: AttributesFormatString=|
      | %<ID>
      | %<Vbase>V
      | %<VLF>pu
      | %<angleLF>deg.
      | %<Name>
  bus508 : powerlib/Measurements/Load Flow Bus  LConnTagsString=a  ID=bus508  Vbase=110000  Vref=1  Vangle=0  VLF=1  angleLF=0
      settings: AttributesFormatString=|
      | %<ID>
      | %<Vbase>V
      | %<VLF>pu
      | %<angleLF>deg.
      | %<Name>
  bus509 : powerlib/Measurements/Load Flow Bus  LConnTagsString=a  ID=bus509  Vbase=110000  Vref=1  Vangle=0  VLF=1  angleLF=0
      settings: AttributesFormatString=|
      | %<ID>
      | %<Vbase>V
      | %<VLF>pu
      | %<angleLF>deg.
      | %<Name>
  bus51 : powerlib/Measurements/Load Flow Bus  LConnTagsString=a  ID=bus51  Vbase=110000  Vref=1  Vangle=0  VLF=1  angleLF=0
      settings: AttributesFormatString=|
      | %<ID>
      | %<Vbase>V
      | %<VLF>pu
      | %<angleLF>deg.
      | %<Name>
  bus510 : powerlib/Measurements/Load Flow Bus  LConnTagsString=a  ID=bus510  Vbase=110000  Vref=1  Vangle=0  VLF=1  angleLF=0
      settings: AttributesFormatString=|
      | %<ID>
      | %<Vbase>V
      | %<VLF>pu
      | %<angleLF>deg.
      | %<Name>
  bus511 : powerlib/Measurements/Load Flow Bus  LConnTagsString=a  ID=bus511  Vbase=110000  Vref=1  Vangle=0  VLF=1  angleLF=0
      settings: AttributesFormatString=|
      | %<ID>
      | %<Vbase>V
      | %<VLF>pu
      | %<angleLF>deg.
      | %<Name>
  bus512 : powerlib/Measurements/Load Flow Bus  LConnTagsString=a  ID=bus512  Vbase=110000  Vref=1  Vangle=0  VLF=1  angleLF=0
      settings: AttributesFormatString=|
      | %<ID>
      | %<Vbase>V
      | %<VLF>pu
      | %<angleLF>deg.
      | %<Name>
  bus513 : powerlib/Measurements/Load Flow Bus  LConnTagsString=a  ID=bus513  Vbase=110000  Vref=1  Vangle=0  VLF=1  angleLF=0
      settings: AttributesFormatString=|
      | %<ID>
      | %<Vbase>V
      | %<VLF>pu
      | %<angleLF>deg.
      | %<Name>
  bus514 : powerlib/Measurements/Load Flow Bus  LConnTagsString=a  ID=bus514  Vbase=110000  Vref=1  Vangle=0  VLF=1  angleLF=0
      settings: AttributesFormatString=|
      | %<ID>
      | %<Vbase>V
      | %<VLF>pu
      | %<angleLF>deg.
      | %<Name>
  bus515 : powerlib/Measurements/Load Flow Bus  LConnTagsString=a  ID=bus515  Vbase=110000  Vref=1  Vangle=0  VLF=1  angleLF=0
      settings: AttributesFormatString=|
      | %<ID>
      | %<Vbase>V
      | %<VLF>pu
      | %<angleLF>deg.
      | %<Name>
  bus516 : powerlib/Measurements/Load Flow Bus  LConnTagsString=a  ID=bus516  Vbase=110000  Vref=1  Vangle=0  VLF=1  angleLF=0
      settings: AttributesFormatString=|
      | %<ID>
      | %<Vbase>V
      | %<VLF>pu
      | %<angleLF>deg.
      | %<Name>
  bus517 : powerlib/Measurements/Load Flow Bus  LConnTagsString=a  ID=bus517  Vbase=110000  Vref=1  Vangle=0  VLF=1  angleLF=0
      settings: AttributesFormatString=|
      | %<ID>
      | %<Vbase>V
      | %<VLF>pu
      | %<angleLF>deg.
      | %<Name>
  bus518 : powerlib/Measurements/Load Flow Bus  LConnTagsString=a  ID=bus518  Vbase=110000  Vref=1  Vangle=0  VLF=1  angleLF=0
      settings: AttributesFormatString=|
      | %<ID>
      | %<Vbase>V
      | %<VLF>pu
      | %<angleLF>deg.
      | %<Name>
  bus519 : powerlib/Measurements/Load Flow Bus  LConnTagsString=a  ID=bus519  Vbase=110000  Vref=1  Vangle=0  VLF=1  angleLF=0
      settings: AttributesFormatString=|
      | %<ID>
      | %<Vbase>V
      | %<VLF>pu
      | %<angleLF>deg.
      | %<Name>
  bus52 : powerlib/Measurements/Load Flow Bus  LConnTagsString=a  ID=bus52  Vbase=110000  Vref=1  Vangle=0  VLF=1  angleLF=0
      settings: AttributesFormatString=|
      | %<ID>
      | %<Vbase>V
      | %<VLF>pu
      | %<angleLF>deg.
      | %<Name>
  bus520 : powerlib/Measurements/Load Flow Bus  LConnTagsString=a  ID=bus520  Vbase=110000  Vref=1  Vangle=0  VLF=1  angleLF=0
      settings: AttributesFormatString=|
      | %<ID>
      | %<Vbase>V
      | %<VLF>pu
      | %<angleLF>deg.
      | %<Name>
  bus521 : powerlib/Measurements/Load Flow Bus  LConnTagsString=a  ID=bus521  Vbase=110000  Vref=1  Vangle=0  VLF=1  angleLF=0
      settings: AttributesFormatString=|
      | %<ID>
      | %<Vbase>V
      | %<VLF>pu
      | %<angleLF>deg.
      | %<Name>
  bus522 : powerlib/Measurements/Load Flow Bus  LConnTagsString=a  ID=bus522  Vbase=110000  Vref=1  Vangle=0  VLF=1  angleLF=0
      settings: AttributesFormatString=|
      | %<ID>
      | %<Vbase>V
      | %<VLF>pu
      | %<angleLF>deg.
      | %<Name>
  bus523 : powerlib/Measurements/Load Flow Bus  LConnTagsString=a  ID=bus523  Vbase=110000  Vref=1  Vangle=0  VLF=1  angleLF=0
      settings: AttributesFormatString=|
      | %<ID>
      | %<Vbase>V
      | %<VLF>pu
      | %<angleLF>deg.
      | %<Name>
  bus524 : powerlib/Measurements/Load Flow Bus  LConnTagsString=a  ID=bus524  Vbase=110000  Vref=1  Vangle=0  VLF=1  angleLF=0
      settings: AttributesFormatString=|
      | %<ID>
      | %<Vbase>V
      | %<VLF>pu
      | %<angleLF>deg.
      | %<Name>
  bus525 : powerlib/Measurements/Load Flow Bus  LConnTagsString=a  ID=bus525  Vbase=400000  Vref=1  Vangle=0  VLF=1  angleLF=0
      settings: AttributesFormatString=|
      | %<ID>
      | %<Vbase>V
      | %<VLF>pu
      | %<angleLF>deg.
      | %<Name>
  bus526 : powerlib/Measurements/Load Flow Bus  LConnTagsString=a  ID=bus526  Vbase=400000  Vref=1  Vangle=0  VLF=1  angleLF=0
      settings: AttributesFormatString=|
      | %<ID>
      | %<Vbase>V
      | %<VLF>pu
      | %<angleLF>deg.
      | %<Name>
  bus527 : powerlib/Measurements/Load Flow Bus  LConnTagsString=a  ID=bus527  Vbase=400000  Vref=1  Vangle=0  VLF=1  angleLF=0
      settings: AttributesFormatString=|
      | %<ID>
      | %<Vbase>V
      | %<VLF>pu
      | %<angleLF>deg.
      | %<Name>
  bus528 : powerlib/Measurements/Load Flow Bus  LConnTagsString=a  ID=bus528  Vbase=400000  Vref=1  Vangle=0  VLF=1  angleLF=0
      settings: AttributesFormatString=|
      | %<ID>
      | %<Vbase>V
      | %<VLF>pu
      | %<angleLF>deg.
      | %<Name>
  bus529 : powerlib/Measurements/Load Flow Bus  LConnTagsString=a  ID=bus529  Vbase=400000  Vref=1  Vangle=0  VLF=1  angleLF=0
      settings: AttributesFormatString=|
      | %<ID>
      | %<Vbase>V
      | %<VLF>pu
      | %<angleLF>deg.
      | %<Name>
  bus53 : powerlib/Measurements/Load Flow Bus  LConnTagsString=a  ID=bus53  Vbase=110000  Vref=1  Vangle=0  VLF=1  angleLF=0
      settings: AttributesFormatString=|
      | %<ID>
      | %<Vbase>V
      | %<VLF>pu
      | %<angleLF>deg.
      | %<Name>
  bus530 : powerlib/Measurements/Load Flow Bus  LConnTagsString=a  ID=bus530  Vbase=400000  Vref=1  Vangle=0  VLF=1  angleLF=0
      settings: AttributesFormatString=|
      | %<ID>
      | %<Vbase>V
      | %<VLF>pu
      | %<angleLF>deg.
      | %<Name>
  bus531 : powerlib/Measurements/Load Flow Bus  LConnTagsString=a  ID=bus531  Vbase=400000  Vref=1  Vangle=0  VLF=1  angleLF=0
      settings: AttributesFormatString=|
      | %<ID>
      | %<Vbase>V
      | %<VLF>pu
      | %<angleLF>deg.
      | %<Name>
  bus532 : powerlib/Measurements/Load Flow Bus  LConnTagsString=a  ID=bus532  Vbase=400000  Vref=1  Vangle=0  VLF=1  angleLF=0
      settings: AttributesFormatString=|
      | %<ID>
      | %<Vbase>V
      | %<VLF>pu
      | %<angleLF>deg.
      | %<Name>
  bus533 : powerlib/Measurements/Load Flow Bus  LConnTagsString=a  ID=bus533  Vbase=400000  Vref=1  Vangle=0  VLF=1  angleLF=0
      settings: AttributesFormatString=|
      | %<ID>
      | %<Vbase>V
      | %<VLF>pu
      | %<angleLF>deg.
      | %<Name>
  bus534 : powerlib/Measurements/Load Flow Bus  LConnTagsString=a  ID=bus534  Vbase=400000  Vref=1  Vangle=0  VLF=1  angleLF=0
      settings: AttributesFormatString=|
      | %<ID>
      | %<Vbase>V
      | %<VLF>pu
      | %<angleLF>deg.
      | %<Name>
  bus54 : powerlib/Measurements/Load Flow Bus  LConnTagsString=a  ID=bus54  Vbase=110000  Vref=1  Vangle=0  VLF=1  angleLF=0
      settings: AttributesFormatString=|
      | %<ID>
      | %<Vbase>V
      | %<VLF>pu
      | %<angleLF>deg.
      | %<Name>
  bus55 : powerlib/Measurements/Load Flow Bus  LConnTagsString=a  ID=bus55  Vbase=110000  Vref=1  Vangle=0  VLF=1  angleLF=0
      settings: AttributesFormatString=|
      | %<ID>
      | %<Vbase>V
      | %<VLF>pu
      | %<angleLF>deg.
      | %<Name>
  bus56 : powerlib/Measurements/Load Flow Bus  LConnTagsString=a  ID=bus56  Vbase=110000  Vref=1  Vangle=0  VLF=1  angleLF=0
      settings: AttributesFormatString=|
      | %<ID>
      | %<Vbase>V
      | %<VLF>pu
      | %<angleLF>deg.
      | %<Name>
  bus57 : powerlib/Measurements/Load Flow Bus  LConnTagsString=a  ID=bus57  Vbase=110000  Vref=1  Vangle=0  VLF=1  angleLF=0
      settings: AttributesFormatString=|
      | %<ID>
      | %<Vbase>V
      | %<VLF>pu
      | %<angleLF>deg.
      | %<Name>
  bus58 : powerlib/Measurements/Load Flow Bus  LConnTagsString=a  ID=bus58  Vbase=110000  Vref=1  Vangle=0  VLF=1  angleLF=0
      settings: AttributesFormatString=|
      | %<ID>
      | %<Vbase>V
      | %<VLF>pu
      | %<angleLF>deg.
      | %<Name>
  bus59 : powerlib/Measurements/Load Flow Bus  LConnTagsString=a  ID=bus59  Vbase=110000  Vref=1  Vangle=0  VLF=1  angleLF=0
      settings: AttributesFormatString=|
      | %<ID>
      | %<Vbase>V
      | %<VLF>pu
      | %<angleLF>deg.
      | %<Name>
  bus6 : powerlib/Measurements/Load Flow Bus  LConnTagsString=a  ID=bus6  Vbase=20000  Vref=1  Vangle=0  VLF=1  angleLF=0
      settings: AttributesFormatString=|
      | %<ID>
      | %<Vbase>V
      | %<VLF>pu
      | %<angleLF>deg.
      | %<Name>
  bus60 : powerlib/Measurements/Load Flow Bus  LConnTagsString=a  ID=bus60  Vbase=110000  Vref=1  Vangle=0  VLF=1  angleLF=0
      settings: AttributesFormatString=|
      | %<ID>
      | %<Vbase>V
      | %<VLF>pu
      | %<angleLF>deg.
      | %<Name>
  bus61 : powerlib/Measurements/Load Flow Bus  LConnTagsString=a  ID=bus61  Vbase=110000  Vref=1  Vangle=0  VLF=1  angleLF=0
      settings: AttributesFormatString=|
      | %<ID>
      | %<Vbase>V
      | %<VLF>pu
      | %<angleLF>deg.
      | %<Name>
  bus62 : powerlib/Measurements/Load Flow Bus  LConnTagsString=a  ID=bus62  Vbase=110000  Vref=1  Vangle=0  VLF=1  angleLF=0
      settings: AttributesFormatString=|
      | %<ID>
      | %<Vbase>V
      | %<VLF>pu
      | %<angleLF>deg.
      | %<Name>
  bus63 : powerlib/Measurements/Load Flow Bus  LConnTagsString=a  ID=bus63  Vbase=110000  Vref=1  Vangle=0  VLF=1  angleLF=0
      settings: AttributesFormatString=|
      | %<ID>
      | %<Vbase>V
      | %<VLF>pu
      | %<angleLF>deg.
      | %<Name>
  bus64 : powerlib/Measurements/Load Flow Bus  LConnTagsString=a  ID=bus64  Vbase=110000  Vref=1  Vangle=0  VLF=1  angleLF=0
      settings: AttributesFormatString=|
      | %<ID>
      | %<Vbase>V
      | %<VLF>pu
      | %<angleLF>deg.
      | %<Name>
  bus65 : powerlib/Measurements/Load Flow Bus  LConnTagsString=a  ID=bus65  Vbase=110000  Vref=1  Vangle=0  VLF=1  angleLF=0
      settings: AttributesFormatString=|
      | %<ID>
      | %<Vbase>V
      | %<VLF>pu
      | %<angleLF>deg.
      | %<Name>
  bus66 : powerlib/Measurements/Load Flow Bus  LConnTagsString=a  ID=bus66  Vbase=110000  Vref=1  Vangle=0  VLF=1  angleLF=0
      settings: AttributesFormatString=|
      | %<ID>
      | %<Vbase>V
      | %<VLF>pu
      | %<angleLF>deg.
      | %<Name>
  bus67 : powerlib/Measurements/Load Flow Bus  LConnTagsString=a  ID=bus67  Vbase=110000  Vref=1  Vangle=0  VLF=1  angleLF=0
      settings: AttributesFormatString=|
      | %<ID>
      | %<Vbase>V
      | %<VLF>pu
      | %<angleLF>deg.
      | %<Name>
  bus68 : powerlib/Measurements/Load Flow Bus  LConnTagsString=a  ID=bus68  Vbase=110000  Vref=1  Vangle=0  VLF=1  angleLF=0
      settings: AttributesFormatString=|
      | %<ID>
      | %<Vbase>V
      | %<VLF>pu
      | %<angleLF>deg.
      | %<Name>
  bus69 : powerlib/Measurements/Load Flow Bus  LConnTagsString=a  ID=bus69  Vbase=110000  Vref=1  Vangle=0  VLF=1  angleLF=0
      settings: AttributesFormatString=|
      | %<ID>
      | %<Vbase>V
      | %<VLF>pu
      | %<angleLF>deg.
      | %<Name>
  bus7 : powerlib/Measurements/Load Flow Bus  LConnTagsString=a  ID=bus7  Vbase=20000  Vref=1  Vangle=0  VLF=1  angleLF=0
      settings: AttributesFormatString=|
      | %<ID>
      | %<Vbase>V
      | %<VLF>pu
      | %<angleLF>deg.
      | %<Name>
  bus70 : powerlib/Measurements/Load Flow Bus  LConnTagsString=a  ID=bus70  Vbase=110000  Vref=1  Vangle=0  VLF=1  angleLF=0
      settings: AttributesFormatString=|
      | %<ID>
      | %<Vbase>V
      | %<VLF>pu
      | %<angleLF>deg.
      | %<Name>
  bus71 : powerlib/Measurements/Load Flow Bus  LConnTagsString=a  ID=bus71  Vbase=110000  Vref=1  Vangle=0  VLF=1  angleLF=0
      settings: AttributesFormatString=|
      | %<ID>
      | %<Vbase>V
      | %<VLF>pu
      | %<angleLF>deg.
      | %<Name>
  bus72 : powerlib/Measurements/Load Flow Bus  LConnTagsString=a  ID=bus72  Vbase=110000  Vref=1  Vangle=0  VLF=1  angleLF=0
      settings: AttributesFormatString=|
      | %<ID>
      | %<Vbase>V
      | %<VLF>pu
      | %<angleLF>deg.
      | %<Name>
  bus73 : powerlib/Measurements/Load Flow Bus  LConnTagsString=a  ID=bus73  Vbase=110000  Vref=1  Vangle=0  VLF=1  angleLF=0
      settings: AttributesFormatString=|
      | %<ID>
      | %<Vbase>V
      | %<VLF>pu
      | %<angleLF>deg.
      | %<Name>
  bus74 : powerlib/Measurements/Load Flow Bus  LConnTagsString=a  ID=bus74  Vbase=110000  Vref=1  Vangle=0  VLF=1  angleLF=0
      settings: AttributesFormatString=|
      | %<ID>
      | %<Vbase>V
      | %<VLF>pu
      | %<angleLF>deg.
      | %<Name>
  bus75 : powerlib/Measurements/Load Flow Bus  LConnTagsString=a  ID=bus75  Vbase=110000  Vref=1  Vangle=0  VLF=1  angleLF=0
      settings: AttributesFormatString=|
      | %<ID>
      | %<Vbase>V
      | %<VLF>pu
      | %<angleLF>deg.
      | %<Name>
  bus76 : powerlib/Measurements/Load Flow Bus  LConnTagsString=a  ID=bus76  Vbase=110000  Vref=1  Vangle=0  VLF=1  angleLF=0
      settings: AttributesFormatString=|
      | %<ID>
      | %<Vbase>V
      | %<VLF>pu
      | %<angleLF>deg.
      | %<Name>
  bus77 : powerlib/Measurements/Load Flow Bus  LConnTagsString=a  ID=bus77  Vbase=110000  Vref=1  Vangle=0  VLF=1  angleLF=0
      settings: AttributesFormatString=|
      | %<ID>
      | %<Vbase>V
      | %<VLF>pu
      | %<angleLF>deg.
      | %<Name>
  bus78 : powerlib/Measurements/Load Flow Bus  LConnTagsString=a  ID=bus78  Vbase=110000  Vref=1  Vangle=0  VLF=1  angleLF=0
      settings: AttributesFormatString=|
      | %<ID>
      | %<Vbase>V
      | %<VLF>pu
      | %<angleLF>deg.
      | %<Name>
  bus79 : powerlib/Measurements/Load Flow Bus  LConnTagsString=a  ID=bus79  Vbase=110000  Vref=1  Vangle=0  VLF=1  angleLF=0
      settings: AttributesFormatString=|
      | %<ID>
      | %<Vbase>V
      | %<VLF>pu
      | %<angleLF>deg.
      | %<Name>
  bus8 : powerlib/Measurements/Load Flow Bus  LConnTagsString=a  ID=bus8  Vbase=20000  Vref=1  Vangle=0  VLF=1  angleLF=0
      settings: AttributesFormatString=|
      | %<ID>
      | %<Vbase>V
      | %<VLF>pu
      | %<angleLF>deg.
      | %<Name>
  bus80 : powerlib/Measurements/Load Flow Bus  LConnTagsString=a  ID=bus80  Vbase=110000  Vref=1  Vangle=0  VLF=1  angleLF=0
      settings: AttributesFormatString=|
      | %<ID>
      | %<Vbase>V
      | %<VLF>pu
      | %<angleLF>deg.
      | %<Name>
  bus81 : powerlib/Measurements/Load Flow Bus  LConnTagsString=a  ID=bus81  Vbase=110000  Vref=1  Vangle=0  VLF=1  angleLF=0
      settings: AttributesFormatString=|
      | %<ID>
      | %<Vbase>V
      | %<VLF>pu
      | %<angleLF>deg.
      | %<Name>
  bus82 : powerlib/Measurements/Load Flow Bus  LConnTagsString=a  ID=bus82  Vbase=110000  Vref=1  Vangle=0  VLF=1  angleLF=0
      settings: AttributesFormatString=|
      | %<ID>
      | %<Vbase>V
      | %<VLF>pu
      | %<angleLF>deg.
      | %<Name>
  bus83 : powerlib/Measurements/Load Flow Bus  LConnTagsString=a  ID=bus83  Vbase=110000  Vref=1  Vangle=0  VLF=1  angleLF=0
      settings: AttributesFormatString=|
      | %<ID>
      | %<Vbase>V
      | %<VLF>pu
      | %<angleLF>deg.
      | %<Name>
  bus84 : powerlib/Measurements/Load Flow Bus  LConnTagsString=a  ID=bus84  Vbase=110000  Vref=1  Vangle=0  VLF=1  angleLF=0
      settings: AttributesFormatString=|
      | %<ID>
      | %<Vbase>V
      | %<VLF>pu
      | %<angleLF>deg.
      | %<Name>
  bus85 : powerlib/Measurements/Load Flow Bus  LConnTagsString=a  ID=bus85  Vbase=110000  Vref=1  Vangle=0  VLF=1  angleLF=0
      settings: AttributesFormatString=|
      | %<ID>
      | %<Vbase>V
      | %<VLF>pu
      | %<angleLF>deg.
      | %<Name>
  bus86 : powerlib/Measurements/Load Flow Bus  LConnTagsString=a  ID=bus86  Vbase=110000  Vref=1  Vangle=0  VLF=1  angleLF=0
      settings: AttributesFormatString=|
      | %<ID>
      | %<Vbase>V
      | %<VLF>pu
      | %<angleLF>deg.
      | %<Name>
  bus87 : powerlib/Measurements/Load Flow Bus  LConnTagsString=a  ID=bus87  Vbase=110000  Vref=1  Vangle=0  VLF=1  angleLF=0
      settings: AttributesFormatString=|
      | %<ID>
      | %<Vbase>V
      | %<VLF>pu
      | %<angleLF>deg.
      | %<Name>
  bus88 : powerlib/Measurements/Load Flow Bus  LConnTagsString=a  ID=bus88  Vbase=110000  Vref=1  Vangle=0  VLF=1  angleLF=0
      settings: AttributesFormatString=|
      | %<ID>
      | %<Vbase>V
      | %<VLF>pu
      | %<angleLF>deg.
      | %<Name>
  bus89 : powerlib/Measurements/Load Flow Bus  LConnTagsString=a  ID=bus89  Vbase=110000  Vref=1  Vangle=0  VLF=1  angleLF=0
      settings: AttributesFormatString=|
      | %<ID>
      | %<Vbase>V
      | %<VLF>pu
      | %<angleLF>deg.
      | %<Name>
  bus9 : powerlib/Measurements/Load Flow Bus  LConnTagsString=a  ID=bus9  Vbase=20000  Vref=1  Vangle=0  VLF=1  angleLF=0
      settings: AttributesFormatString=|
      | %<ID>
      | %<Vbase>V
      | %<VLF>pu
      | %<angleLF>deg.
      | %<Name>
  bus90 : powerlib/Measurements/Load Flow Bus  LConnTagsString=a  ID=bus90  Vbase=110000  Vref=1  Vangle=0  VLF=1  angleLF=0
      settings: AttributesFormatString=|
      | %<ID>
      | %<Vbase>V
      | %<VLF>pu
      | %<angleLF>deg.
      | %<Name>
  bus91 : powerlib/Measurements/Load Flow Bus  LConnTagsString=a  ID=bus91  Vbase=110000  Vref=1  Vangle=0  VLF=1  angleLF=0
      settings: AttributesFormatString=|
      | %<ID>
      | %<Vbase>V
      | %<VLF>pu
      | %<angleLF>deg.
      | %<Name>
  bus92 : powerlib/Measurements/Load Flow Bus  LConnTagsString=a  ID=bus92  Vbase=110000  Vref=1  Vangle=0  VLF=1  angleLF=0
      settings: AttributesFormatString=|
      | %<ID>
      | %<Vbase>V
      | %<VLF>pu
      | %<angleLF>deg.
      | %<Name>
  bus93 : powerlib/Measurements/Load Flow Bus  LConnTagsString=a  ID=bus93  Vbase=110000  Vref=1  Vangle=0  VLF=1  angleLF=0
      settings: AttributesFormatString=|
      | %<ID>
      | %<Vbase>V
      | %<VLF>pu
      | %<angleLF>deg.
      | %<Name>
  bus94 : powerlib/Measurements/Load Flow Bus  LConnTagsString=a  ID=bus94  Vbase=110000  Vref=1  Vangle=0  VLF=1  angleLF=0
      settings: AttributesFormatString=|
      | %<ID>
      | %<Vbase>V
      | %<VLF>pu
      | %<angleLF>deg.
      | %<Name>
  bus95 : powerlib/Measurements/Load Flow Bus  LConnTagsString=a  ID=bus95  Vbase=110000  Vref=1  Vangle=0  VLF=1  angleLF=0
      settings: AttributesFormatString=|
      | %<ID>
      | %<Vbase>V
      | %<VLF>pu
      | %<angleLF>deg.
      | %<Name>
  bus96 : powerlib/Measurements/Load Flow Bus  LConnTagsString=a  ID=bus96  Vbase=110000  Vref=1  Vangle=0  VLF=1  angleLF=0
      settings: AttributesFormatString=|
      | %<ID>
      | %<Vbase>V
      | %<VLF>pu
      | %<angleLF>deg.
      | %<Name>
  bus97 : powerlib/Measurements/Load Flow Bus  LConnTagsString=a  ID=bus97  Vbase=110000  Vref=1  Vangle=0  VLF=1  angleLF=0
      settings: AttributesFormatString=|
      | %<ID>
      | %<Vbase>V
      | %<VLF>pu
      | %<angleLF>deg.
      | %<Name>
  bus98 : powerlib/Measurements/Load Flow Bus  LConnTagsString=a  ID=bus98  Vbase=110000  Vref=1  Vangle=0  VLF=1  angleLF=0
      settings: AttributesFormatString=|
      | %<ID>
      | %<Vbase>V
      | %<VLF>pu
      | %<angleLF>deg.
      | %<Name>
  bus99 : powerlib/Measurements/Load Flow Bus  LConnTagsString=a  ID=bus99  Vbase=110000  Vref=1  Vangle=0  VLF=1  angleLF=0
      settings: AttributesFormatString=|
      | %<ID>
      | %<Vbase>V
      | %<VLF>pu
      | %<angleLF>deg.
      | %<Name>
  powergui : powerlib/powergui  Priority=1  SimulationMode=Continuous  SolverType=Tustin  SampleTime=50e-6  frequency=60  SPID=off  DisableSnubberDevices=off  DisableRonSwitches=off  DisableVfSwitches=off  SwTol=0  Interpol=off  DisplayEquations=off  Ts=0  methode=off  frequencyindice=60  Pbase=100e6  ErrMax=1e-4  Iterations=50  UnitsV=kV  UnitsW=MW  FunctionMessages=off  echomessages=off  HookPort=off  EnableUseOfTLC=off  x0status=blocks  RestoreLinks=warning  ResistiveCurrentMeasurement=off  Frange=[0:2:500]  Ylog=off  Xlog=on  ShowGrid=off  save=off  variable=ZData  structure=0  ZoomFFT=off  StartTime=0.0  cycles=1  DisplayStyle=1  fundamental=60  FreqAxis=off  MaxFrequency=1000  frequencyindicesteady=1  RmsSteady=1  display=off
  Ötztal___Zirl_CN_147563007_110000_CN_100404264_110000 : powerlib/Elements/Distributed Parameters Line  Phases=3  Frequency=60  Resistance=[0.01273 0.3864]  Inductance="[0.9337e-3  4.1264e-3]"  Capacitance=[12.74e-9 7.751e-9]  Length=100  x1=[0 0 0 0; 0.0001244 0 0 0; 0.0002488 0 0 0; 0.0003733 0 0 0; 0.0004977 0 0 0; 0.0006221 0 0 0]  x2=[0 0 0 0; 0.0001244 0 0 0; 0.0002488 0 0 0; 0.0003733 0 0 0; 0.0004977 0 0 0; 0.0006221 0 0 0]  x3=[0 0 0 0; 0.0001244 0 0 0; 0.0002488 0 0 0; 0.0003733 0 0 0; 0.0004977 0 0 0; 0.0006221 0 0 0]  x4=[0 0 0 0; 0.0001244 0 0 0; 0.0002488 0 0 0; 0.0003733 0 0 0; 0.0004977 0 0 0; 0.0006221 0 0 0]  x5=0  V1=ones(3,3)  V2=ones(3,3)  I1=ones(3,3)  I2=ones(3,3)  nHarmo=1  Measurements=None
  connections:
  T_88379010_220000;110000_/LConn1 -- _CN_88379010_20000_CN_119130475_20000/LConn1
  T_88379010_220000;110000_/LConn2 -- _CN_88379010_20000_CN_119130475_20000/LConn2
  _CN_88379010_20000_CN_119130475_20000/LConn3 -- T_88379010_220000;110000_/LConn3 -- bus1/LConn1
  _CN_88379010_20000_CN_119130475_20000/RConn1 -- T_119130475_220000;110000_/RConn1 -- _CN_103428598_20000_CN_119130475_20000/LConn1 -- L_119130475/LConn1
  _CN_88379010_20000_CN_119130475_20000/RConn2 -- T_119130475_220000;110000_/RConn2 -- _CN_103428598_20000_CN_119130475_20000/LConn2 -- L_119130475/LConn2
  _CN_88379010_20000_CN_119130475_20000/RConn3 -- T_119130475_220000;110000_/RConn3 -- _CN_103428598_20000_CN_119130475_20000/LConn3 -- L_119130475/LConn3 -- bus2/LConn1
  _CN_173431812_20000_CN_33691043_20000/LConn1 -- T_173431812_220000;110000_/RConn1 -- L_173431812/LConn1
  _CN_173431812_20000_CN_33691043_20000/LConn2 -- T_173431812_220000;110000_/RConn2 -- L_173431812/LConn2
  _CN_173431812_20000_CN_33691043_20000/LConn3 -- T_173431812_220000;110000_/RConn3 -- L_173431812/LConn3 -- bus3/LConn1
  _CN_173431812_20000_CN_33691043_20000/RConn1 -- T_33691043_220000;110000_/LConn1 -- _CN_33691043_20000_CN_136068907_20000/LConn1 -- _CN_33691043_20000_CN_149965738_20000/LConn1 -- _CN_33691043_20000_CN_169057271_20000/LConn1
  _CN_173431812_20000_CN_33691043_20000/RConn2 -- T_33691043_220000;110000_/LConn2 -- _CN_33691043_20000_CN_136068907_20000/LConn2 -- _CN_33691043_20000_CN_149965738_20000/LConn2 -- _CN_33691043_20000_CN_169057271_20000/LConn2
  _CN_173431812_20000_CN_33691043_20000/RConn3 -- T_33691043_220000;110000_/LConn3 -- _CN_33691043_20000_CN_136068907_20000/LConn3 -- _CN_33691043_20000_CN_149965738_20000/LConn3 -- _CN_33691043_20000_CN_169057271_20000/LConn3 -- bus4/LConn1
  T_150282502_220000_/LConn1 -- _CN_150282502_20000_CN_194462560_20000/LConn1
  T_150282502_220000_/LConn2 -- _CN_150282502_20000_CN_194462560_20000/LConn2
  _CN_150282502_20000_CN_194462560_20000/LConn3 -- T_150282502_220000_/LConn3 -- bus5/LConn1
  G_194462560_Kanteleen_Voima_Oy_Haapaveden_voimalaitos/RConn1 -- _CN_150282502_20000_CN_194462560_20000/RConn1
  G_194462560_Kanteleen_Voima_Oy_Haapaveden_voimalaitos/RConn2 -- _CN_150282502_20000_CN_194462560_20000/RConn2
  _CN_150282502_20000_CN_194462560_20000/RConn3 -- G_194462560_Kanteleen_Voima_Oy_Haapaveden_voimalaitos/RConn3 -- bus6/LConn1
  _CN_314853393_20000_CN_391145068_20000/LConn1 -- T_314853393_220000;110000_/LConn1 -- _CN_314853393_20000_CN_55609623_20000/LConn1
  _CN_314853393_20000_CN_391145068_20000/LConn2 -- T_314853393_220000;110000_/LConn2 -- _CN_314853393_20000_CN_55609623_20000/LConn2
  _CN_314853393_20000_CN_391145068_20000/LConn3 -- T_314853393_220000;110000_/LConn3 -- _CN_314853393_20000_CN_55609623_20000/LConn3 -- bus7/LConn1
  _CN_314853393_20000_CN_391145068_20000/RConn1 -- T_391145068_220000;110000_/LConn1 -- _CN_379937972_20000_CN_391145068_20000/LConn1 -- _CN_391145068_20000_CN_391142388_20000/LConn1
  _CN_314853393_20000_CN_391145068_20000/RConn2 -- T_391145068_220000;110000_/LConn2 -- _CN_379937972_20000_CN_391145068_20000/LConn2 -- _CN_391145068_20000_CN_391142388_20000/LConn2
  _CN_314853393_20000_CN_391145068_20000/RConn3 -- T_391145068_220000;110000_/LConn3 -- _CN_379937972_20000_CN_391145068_20000/LConn3 -- _CN_391145068_20000_CN_391142388_20000/LConn3 -- bus8/LConn1
  _CN_314853393_20000_CN_55609623_20000/RConn1 -- T_55609623_220000;110000_/LConn1 -- _CN_286955411_20000_CN_55609623_20000/LConn1
  _CN_314853393_20000_CN_55609623_20000/RConn2 -- T_55609623_220000;110000_/LConn2 -- _CN_286955411_20000_CN_55609623_20000/LConn2
  _CN_314853393_20000_CN_55609623_20000/RConn3 -- T_55609623_220000;110000_/LConn3 -- _CN_286955411_20000_CN_55609623_20000/LConn3 -- bus9/LConn1
  T_391142034_220000_/LConn1 -- _CN_391142034_20000_CN_388655178_20000/LConn1
  T_391142034_220000_/LConn2 -- _CN_391142034_20000_CN_388655178_20000/LConn2
  _CN_391142034_20000_CN_388655178_20000/LConn3 -- T_391142034_220000_/LConn3 -- bus10/LConn1
  _CN_391142034_20000_CN_388655178_20000/RConn1 -- T_388655178_400000;220000;110000_/RConn1 -- _CN_388655178_20000_CN_391142388_20000/LConn1 -- L_388655178/LConn1
  _CN_391142034_20000_CN_388655178_20000/RConn2 -- T_388655178_400000;220000;110000_/RConn2 -- _CN_388655178_20000_CN_391142388_20000/LConn2 -- L_388655178/LConn2
  _CN_391142034_20000_CN_388655178_20000/RConn3 -- T_388655178_400000;220000;110000_/RConn3 -- _CN_388655178_20000_CN_391142388_20000/LConn3 -- L_388655178/LConn3 -- bus11/LConn1
  _CN_286955411_20000_CN_388832477_20000/LConn1 -- T_286955411_220000_/LConn1 -- _CN_286955411_20000_CN_55609623_20000/RConn1
  _CN_286955411_20000_CN_388832477_20000/LConn2 -- T_286955411_220000_/LConn2 -- _CN_286955411_20000_CN_55609623_20000/RConn2
  _CN_286955411_20000_CN_388832477_20000/LConn3 -- T_286955411_220000_/LConn3 -- _CN_286955411_20000_CN_55609623_20000/RConn3 -- bus12/LConn1
  _CN_286955411_20000_CN_388832477_20000/RConn1 -- T_388832477_220000_Ossauskoski/LConn1 -- _CN_388832477_20000_CN_213581343_20000/LConn1 -- _CN_388832477_20000_CN_169899622_20000/LConn1
  _CN_286955411_20000_CN_388832477_20000/RConn2 -- T_388832477_220000_Ossauskoski/LConn2 -- _CN_388832477_20000_CN_213581343_20000/LConn2 -- _CN_388832477_20000_CN_169899622_20000/LConn2
  _CN_286955411_20000_CN_388832477_20000/RConn3 -- T_388832477_220000_Ossauskoski/LConn3 -- _CN_388832477_20000_CN_213581343_20000/LConn3 -- _CN_388832477_20000_CN_169899622_20000/LConn3 -- bus13/LConn1
  T_400567451_220000_/LConn1 -- _CN_400567451_20000_CN_379937972_20000/LConn1
  T_400567451_220000_/LConn2 -- _CN_400567451_20000_CN_379937972_20000/LConn2
  _CN_400567451_20000_CN_379937972_20000/LConn3 -- T_400567451_220000_/LConn3 -- bus14/LConn1
  _CN_400567451_20000_CN_379937972_20000/RConn1 -- T_379937972_220000_/RConn1 -- _CN_379937972_20000_CN_391145068_20000/RConn1 -- L_379937972/LConn1
  _CN_400567451_20000_CN_379937972_20000/RConn2 -- T_379937972_220000_/RConn2 -- _CN_379937972_20000_CN_391145068_20000/RConn2 -- L_379937972/LConn2
  _CN_400567451_20000_CN_379937972_20000/RConn3 -- T_379937972_220000_/RConn3 -- _CN_379937972_20000_CN_391145068_20000/RConn3 -- L_379937972/LConn3 -- bus15/LConn1
  _CN_33691043_20000_CN_136068907_20000/RConn1 -- T_136068907_400000;220000;110000_/RConn4 -- L_136068907/LConn1
  _CN_33691043_20000_CN_136068907_20000/RConn2 -- T_136068907_400000;220000;110000_/RConn5 -- L_136068907/LConn2
  _CN_33691043_20000_CN_136068907_20000/RConn3 -- T_136068907_400000;220000;110000_/RConn6 -- L_136068907/LConn3 -- bus16/LConn1
  _CN_33691043_20000_CN_149965738_20000/RConn1 -- T_149965738_220000_/LConn1 -- _CN_149965738_20000_CN_169057271_20000/LConn1 -- _CN_149965738_20000_CN_169057270_20000/LConn1 -- _CN_149965738_20000_CN_149965688_20000/LConn1
  _CN_33691043_20000_CN_149965738_20000/RConn2 -- T_149965738_220000_/LConn2 -- _CN_149965738_20000_CN_169057271_20000/LConn2 -- _CN_149965738_20000_CN_169057270_20000/LConn2 -- _CN_149965738_20000_CN_149965688_20000/LConn2
  _CN_33691043_20000_CN_149965738_20000/RConn3 -- T_149965738_220000_/LConn3 -- _CN_149965738_20000_CN_169057271_20000/LConn3 -- _CN_149965738_20000_CN_169057270_20000/LConn3 -- bus17/LConn1 -- _CN_149965738_20000_CN_149965688_20000/LConn3
  _CN_33691043_20000_CN_169057271_20000/RConn1 -- T_169057271_220000_/LConn1 -- _CN_363178756_20000_CN_169057271_20000/LConn1 -- _CN_149965738_20000_CN_169057271_20000/RConn1
  _CN_33691043_20000_CN_169057271_20000/RConn2 -- T_169057271_220000_/LConn2 -- _CN_363178756_20000_CN_169057271_20000/LConn2 -- _CN_149965738_20000_CN_169057271_20000/RConn2
  _CN_33691043_20000_CN_169057271_20000/RConn3 -- T_169057271_220000_/LConn3 -- _CN_363178756_20000_CN_169057271_20000/LConn3 -- bus18/LConn1 -- _CN_149965738_20000_CN_169057271_20000/RConn3
  G_149965688_Leppiniemi/RConn1 -- _CN_149965738_20000_CN_149965688_20000/RConn1
  G_149965688_Leppiniemi/RConn2 -- _CN_149965738_20000_CN_149965688_20000/RConn2
  _CN_149965738_20000_CN_149965688_20000/RConn3 -- G_149965688_Leppiniemi/RConn3 -- bus19/LConn1
  T_169057270_220000_/LConn1 -- _CN_149965738_20000_CN_169057270_20000/RConn1
  T_169057270_220000_/LConn2 -- _CN_149965738_20000_CN_169057270_20000/RConn2
  _CN_149965738_20000_CN_169057270_20000/RConn3 -- T_169057270_220000_/LConn3 -- bus20/LConn1
  _CN_150209972_20000_CN_103428598_20000/LConn1 -- T_150209972_400000;110000_Tuovila/RConn4 -- _CN_150209972_20000_CN_40644756_20000/LConn1 -- L_150209972/LConn1
  _CN_150209972_20000_CN_103428598_20000/LConn2 -- T_150209972_400000;110000_Tuovila/RConn5 -- _CN_150209972_20000_CN_40644756_20000/LConn2 -- L_150209972/LConn2
  _CN_150209972_20000_CN_103428598_20000/LConn3 -- T_150209972_400000;110000_Tuovila/RConn6 -- _CN_150209972_20000_CN_40644756_20000/LConn3 -- L_150209972/LConn3 -- bus21/LConn1
  _CN_150209972_20000_CN_103428598_20000/RConn1 -- T_103428598_220000;110000_/RConn1 -- _CN_103428598_20000_CN_119130475_20000/RConn1 -- L_103428598/LConn1
  _CN_150209972_20000_CN_103428598_20000/RConn2 -- T_103428598_220000;110000_/RConn2 -- _CN_103428598_20000_CN_119130475_20000/RConn2 -- L_103428598/LConn2
  _CN_150209972_20000_CN_103428598_20000/RConn3 -- T_103428598_220000;110000_/RConn3 -- _CN_103428598_20000_CN_119130475_20000/RConn3 -- L_103428598/LConn3 -- bus22/LConn1
  G_40644756_/RConn1 -- _CN_150209972_20000_CN_40644756_20000/RConn1
  G_40644756_/RConn2 -- _CN_150209972_20000_CN_40644756_20000/RConn2
  _CN_150209972_20000_CN_40644756_20000/RConn3 -- G_40644756_/RConn3 -- bus23/LConn1
  _CN_388655178_20000_CN_391142388_20000/RConn1 -- T_391142388_220000;110000_/RConn1 -- _CN_391145068_20000_CN_391142388_20000/RConn1 -- L_391142388/LConn1
  _CN_388655178_20000_CN_391142388_20000/RConn2 -- T_391142388_220000;110000_/RConn2 -- _CN_391145068_20000_CN_391142388_20000/RConn2 -- L_391142388/LConn2
  _CN_388655178_20000_CN_391142388_20000/RConn3 -- T_391142388_220000;110000_/RConn3 -- _CN_391145068_20000_CN_391142388_20000/RConn3 -- L_391142388/LConn3 -- bus24/LConn1
  _CN_363178756_20000_CN_169057271_20000/RConn1 -- T_363178756_220000;110000_/RConn1 -- L_363178756/LConn1
  _CN_363178756_20000_CN_169057271_20000/RConn2 -- T_363178756_220000;110000_/RConn2 -- L_363178756/LConn2
  _CN_363178756_20000_CN_169057271_20000/RConn3 -- T_363178756_220000;110000_/RConn3 -- L_363178756/LConn3 -- bus25/LConn1
  G_213581343_Tuuliwatti_Tervola_Varevaara/RConn1 -- _CN_388832477_20000_CN_213581343_20000/RConn1
  G_213581343_Tuuliwatti_Tervola_Varevaara/RConn2 -- _CN_388832477_20000_CN_213581343_20000/RConn2
  _CN_388832477_20000_CN_213581343_20000/RConn3 -- G_213581343_Tuuliwatti_Tervola_Varevaara/RConn3 -- bus26/LConn1
  _CN_388832477_20000_CN_169899622_20000/RConn1 -- T_169899622_220000;110000_/RConn1 -- _CN_169899622_20000_CN_169899620_20000/LConn1 -- L_169899622/LConn1
  _CN_388832477_20000_CN_169899622_20000/RConn2 -- T_169899622_220000;110000_/RConn2 -- _CN_169899622_20000_CN_169899620_20000/LConn2 -- L_169899622/LConn2
  _CN_388832477_20000_CN_169899622_20000/RConn3 -- T_169899622_220000;110000_/RConn3 -- _CN_169899622_20000_CN_169899620_20000/LConn3 -- L_169899622/LConn3 -- bus27/LConn1
  _CN_169899622_20000_CN_169899620_20000/RConn1 -- G_169899620_/RConn1 -- _CN_169899622_110000_CN_169899620_20000/LConn1
  _CN_169899622_20000_CN_169899620_20000/RConn2 -- G_169899620_/RConn2 -- _CN_169899622_110000_CN_169899620_20000/LConn2
  _CN_169899622_20000_CN_169899620_20000/RConn3 -- G_169899620_/RConn3 -- _CN_169899622_110000_CN_169899620_20000/LConn3 -- bus28/LConn1
  T_75612161_110000_/LConn1 -- _CN_75612161_110000_CN_144832705_110000/LConn1
  T_75612161_110000_/LConn2 -- _CN_75612161_110000_CN_144832705_110000/LConn2
  _CN_75612161_110000_CN_144832705_110000/LConn3 -- T_75612161_110000_/LConn3 -- bus29/LConn1
  _CN_75612161_110000_CN_144832705_110000/RConn1 -- T_144832705_400000;110000_/RConn1 -- L_144832705/LConn1
  _CN_75612161_110000_CN_144832705_110000/RConn2 -- T_144832705_400000;110000_/RConn2 -- L_144832705/LConn2
  _CN_75612161_110000_CN_144832705_110000/RConn3 -- T_144832705_400000;110000_/RConn3 -- L_144832705/LConn3 -- bus30/LConn1
  T_28604436_110000_Suvilahti/LConn1 -- _CN_28604436_110000_CN_6268760_110000/LConn1
  T_28604436_110000_Suvilahti/LConn2 -- _CN_28604436_110000_CN_6268760_110000/LConn2
  _CN_28604436_110000_CN_6268760_110000/LConn3 -- T_28604436_110000_Suvilahti/LConn3 -- bus31/LConn1
  _CN_28604436_110000_CN_6268760_110000/RConn1 -- T_6268760_110000_Herttoniemi/LConn1 -- _CN_36977363_110000_CN_6268760_110000/LConn1 -- _CN_26331359_110000_CN_6268760_110000/LConn1
  _CN_28604436_110000_CN_6268760_110000/RConn2 -- T_6268760_110000_Herttoniemi/LConn2 -- _CN_36977363_110000_CN_6268760_110000/LConn2 -- _CN_26331359_110000_CN_6268760_110000/LConn2
  _CN_28604436_110000_CN_6268760_110000/RConn3 -- T_6268760_110000_Herttoniemi/LConn3 -- _CN_36977363_110000_CN_6268760_110000/LConn3 -- bus32/LConn1 -- _CN_26331359_110000_CN_6268760_110000/LConn3
  T_232208451__/LConn1 -- _CN_232208451_110000_CN_208979069_110000/LConn1
  T_232208451__/LConn2 -- _CN_232208451_110000_CN_208979069_110000/LConn2
  _CN_232208451_110000_CN_208979069_110000/LConn3 -- T_232208451__/LConn3 -- bus33/LConn1
  _CN_232208451_110000_CN_208979069_110000/RConn1 -- T_208979069_400000;110000_/RConn1 -- _CN_151583286_110000_CN_208979069_110000/LConn1 -- _CN_220230343_110000_CN_208979069_110000/LConn1 -- L_208979069/LConn1
  _CN_232208451_110000_CN_208979069_110000/RConn2 -- T_208979069_400000;110000_/RConn2 -- _CN_151583286_110000_CN_208979069_110000/LConn2 -- _CN_220230343_110000_CN_208979069_110000/LConn2 -- L_208979069/LConn2
  _CN_232208451_110000_CN_208979069_110000/RConn3 -- T_208979069_400000;110000_/RConn3 -- _CN_151583286_110000_CN_208979069_110000/LConn3 -- _CN_220230343_110000_CN_208979069_110000/LConn3 -- L_208979069/LConn3 -- bus34/LConn1
  _CN_187430983_110000_CN_209207437_110000/LConn1 -- T_187430983_110000_/LConn1 -- _CN_187430983_110000_CN_187428237_110000/LConn1
  _CN_187430983_110000_CN_209207437_110000/LConn2 -- T_187430983_110000_/LConn2 -- _CN_187430983_110000_CN_187428237_110000/LConn2
  _CN_187430983_110000_CN_209207437_110000/LConn3 -- T_187430983_110000_/LConn3 -- _CN_187430983_110000_CN_187428237_110000/LConn3 -- bus35/LConn1
  T_209207437_110000_/LConn1 -- _CN_187430983_110000_CN_209207437_110000/RConn1
  T_209207437_110000_/LConn2 -- _CN_187430983_110000_CN_209207437_110000/RConn2
  _CN_187430983_110000_CN_209207437_110000/RConn3 -- T_209207437_110000_/LConn3 -- bus36/LConn1
  T_187428237_110000_/LConn1 -- _CN_187430983_110000_CN_187428237_110000/RConn1
  T_187428237_110000_/LConn2 -- _CN_187430983_110000_CN_187428237_110000/RConn2
  _CN_187430983_110000_CN_187428237_110000/RConn3 -- T_187428237_110000_/LConn3 -- bus37/LConn1
  T_128571465__/LConn1 -- _CN_128571465_110000_CN_128571463_110000/LConn1
  T_128571465__/LConn2 -- _CN_128571465_110000_CN_128571463_110000/LConn2
  _CN_128571465_110000_CN_128571463_110000/LConn3 -- T_128571465__/LConn3 -- bus38/LConn1
  _CN_128571465_110000_CN_128571463_110000/RConn1 -- T_128571463_110000_/LConn1 -- _CN_148312425_110000_CN_128571463_110000/LConn1 -- _CN_197245741_110000_CN_128571463_110000/LConn1
  _CN_128571465_110000_CN_128571463_110000/RConn2 -- T_128571463_110000_/LConn2 -- _CN_148312425_110000_CN_128571463_110000/LConn2 -- _CN_197245741_110000_CN_128571463_110000/LConn2
  _CN_128571465_110000_CN_128571463_110000/RConn3 -- T_128571463_110000_/LConn3 -- _CN_148312425_110000_CN_128571463_110000/LConn3 -- _CN_197245741_110000_CN_128571463_110000/LConn3 -- bus39/LConn1
  _CN_42594389_110000_CN_285480163_110000/LConn1 -- T_42594389_110000_Kangasvuoren_sähköasema/LConn1 -- _CN_42594389_110000_CN_87670572_110000/LConn1 -- _CN_42594389_110000_CN_59014204_110000/LConn1 -- _CN_42594389_110000_CN_43143343_110000/LConn1
  _CN_42594389_110000_CN_285480163_110000/LConn2 -- T_42594389_110000_Kangasvuoren_sähköasema/LConn2 -- _CN_42594389_110000_CN_87670572_110000/LConn2 -- _CN_42594389_110000_CN_59014204_110000/LConn2 -- _CN_42594389_110000_CN_43143343_110000/LConn2
  _CN_42594389_110000_CN_285480163_110000/LConn3 -- T_42594389_110000_Kangasvuoren_sähköasema/LConn3 -- _CN_42594389_110000_CN_87670572_110000/LConn3 -- _CN_42594389_110000_CN_59014204_110000/LConn3 -- _CN_42594389_110000_CN_43143343_110000/LConn3 -- bus40/LConn1
  T_285480163__/LConn1 -- _CN_42594389_110000_CN_285480163_110000/RConn1
  T_285480163__/LConn2 -- _CN_42594389_110000_CN_285480163_110000/RConn2
  _CN_42594389_110000_CN_285480163_110000/RConn3 -- T_285480163__/LConn3 -- bus41/LConn1
  _CN_42594389_110000_CN_87670572_110000/RConn1 -- T_87670572_110000_/LConn1 -- _CN_87670542_110000_CN_87670572_110000/LConn1
  _CN_42594389_110000_CN_87670572_110000/RConn2 -- T_87670572_110000_/LConn2 -- _CN_87670542_110000_CN_87670572_110000/LConn2
  _CN_42594389_110000_CN_87670572_110000/RConn3 -- T_87670572_110000_/LConn3 -- _CN_87670542_110000_CN_87670572_110000/LConn3 -- bus42/LConn1
  _CN_42594389_110000_CN_59014204_110000/RConn1 -- T_59014204__Hämeenlahden_sähköasema/LConn1 -- _CN_59014204_110000_CN_32910454_110000/LConn1 -- _CN_169018002_110000_CN_59014204_110000/LConn1
  _CN_42594389_110000_CN_59014204_110000/RConn2 -- T_59014204__Hämeenlahden_sähköasema/LConn2 -- _CN_59014204_110000_CN_32910454_110000/LConn2 -- _CN_169018002_110000_CN_59014204_110000/LConn2
  _CN_42594389_110000_CN_59014204_110000/RConn3 -- T_59014204__Hämeenlahden_sähköasema/LConn3 -- _CN_59014204_110000_CN_32910454_110000/LConn3 -- bus43/LConn1 -- _CN_169018002_110000_CN_59014204_110000/LConn3
  _CN_42594389_110000_CN_43143343_110000/RConn1 -- T_43143343__/RConn1 -- _CN_43143343_110000_CN_186886932_110000/LConn1 -- _CN_43143343_110000_CN_128255187_110000/LConn1 -- L_43143343/LConn1
  _CN_42594389_110000_CN_43143343_110000/RConn2 -- T_43143343__/RConn2 -- _CN_43143343_110000_CN_186886932_110000/LConn2 -- _CN_43143343_110000_CN_128255187_110000/LConn2 -- L_43143343/LConn2
  _CN_42594389_110000_CN_43143343_110000/RConn3 -- T_43143343__/RConn3 -- _CN_43143343_110000_CN_186886932_110000/LConn3 -- _CN_43143343_110000_CN_128255187_110000/LConn3 -- L_43143343/LConn3 -- bus44/LConn1
  T_151998558_110000_/LConn1 -- _CN_151998558_110000_CN_159153725_110000/LConn1
  T_151998558_110000_/LConn2 -- _CN_151998558_110000_CN_159153725_110000/LConn2
  _CN_151998558_110000_CN_159153725_110000/LConn3 -- T_151998558_110000_/LConn3 -- bus45/LConn1
  T_159153725__/LConn1 -- _CN_151998558_110000_CN_159153725_110000/RConn1
  T_159153725__/LConn2 -- _CN_151998558_110000_CN_159153725_110000/RConn2
  _CN_151998558_110000_CN_159153725_110000/RConn3 -- T_159153725__/LConn3 -- bus46/LConn1
  T_27175012__/LConn1 -- _CN_27175012_110000_CN_108980081_110000/LConn1
  T_27175012__/LConn2 -- _CN_27175012_110000_CN_108980081_110000/LConn2
  _CN_27175012_110000_CN_108980081_110000/LConn3 -- T_27175012__/LConn3 -- bus47/LConn1
  _CN_27175012_110000_CN_108980081_110000/RConn1 -- T_108980081_110000_/LConn1 -- _CN_178307639_110000_CN_108980081_110000/LConn1 -- _CN_159532385_110000_CN_108980081_110000/LConn1
  _CN_27175012_110000_CN_108980081_110000/RConn2 -- T_108980081_110000_/LConn2 -- _CN_178307639_110000_CN_108980081_110000/LConn2 -- _CN_159532385_110000_CN_108980081_110000/LConn2
  _CN_27175012_110000_CN_108980081_110000/RConn3 -- T_108980081_110000_/LConn3 -- _CN_178307639_110000_CN_108980081_110000/LConn3 -- _CN_159532385_110000_CN_108980081_110000/LConn3 -- bus48/LConn1
  T_178370665__/LConn1 -- _CN_178370665_110000_CN_26358836_110000/LConn1
  T_178370665__/LConn2 -- _CN_178370665_110000_CN_26358836_110000/LConn2
  _CN_178370665_110000_CN_26358836_110000/LConn3 -- T_178370665__/LConn3 -- bus49/LConn1
  T_26358836_110000_/LConn1 -- _CN_178370665_110000_CN_26358836_110000/RConn1
  T_26358836_110000_/LConn2 -- _CN_178370665_110000_CN_26358836_110000/RConn2
  _CN_178370665_110000_CN_26358836_110000/RConn3 -- T_26358836_110000_/LConn3 -- bus50/LConn1
  _CN_29421693_110000_CN_169259235_110000/LConn1 -- T_29421693_110000_/LConn1 -- _CN_29421693_110000_CN_130331348_110000/LConn1
  _CN_29421693_110000_CN_169259235_110000/LConn2 -- T_29421693_110000_/LConn2 -- _CN_29421693_110000_CN_130331348_110000/LConn2
  _CN_29421693_110000_CN_169259235_110000/LConn3 -- T_29421693_110000_/LConn3 -- _CN_29421693_110000_CN_130331348_110000/LConn3 -- bus51/LConn1
  T_169259235__/LConn1 -- _CN_29421693_110000_CN_169259235_110000/RConn1
  T_169259235__/LConn2 -- _CN_29421693_110000_CN_169259235_110000/RConn2
  _CN_29421693_110000_CN_169259235_110000/RConn3 -- T_169259235__/LConn3 -- bus52/LConn1
  _CN_29421693_110000_CN_130331348_110000/RConn1 -- T_130331348_110000_/LConn1 -- _CN_130331348_110000_CN_150204241_110000/LConn1
  _CN_29421693_110000_CN_130331348_110000/RConn2 -- T_130331348_110000_/LConn2 -- _CN_130331348_110000_CN_150204241_110000/LConn2
  _CN_29421693_110000_CN_130331348_110000/RConn3 -- T_130331348_110000_/LConn3 -- _CN_130331348_110000_CN_150204241_110000/LConn3 -- bus53/LConn1
  _CN_352399506_110000_CN_136370546_110000/LConn1 -- T_352399506_110000_/LConn1 -- _CN_352399506_110000_CN_103428598_110000/LConn1
  _CN_352399506_110000_CN_136370546_110000/LConn2 -- T_352399506_110000_/LConn2 -- _CN_352399506_110000_CN_103428598_110000/LConn2
  _CN_352399506_110000_CN_136370546_110000/LConn3 -- T_352399506_110000_/LConn3 -- _CN_352399506_110000_CN_103428598_110000/LConn3 -- bus54/LConn1
  T_136370546_110000_/LConn1 -- _CN_352399506_110000_CN_136370546_110000/RConn1
  T_136370546_110000_/LConn2 -- _CN_352399506_110000_CN_136370546_110000/RConn2
  _CN_352399506_110000_CN_136370546_110000/RConn3 -- T_136370546_110000_/LConn3 -- bus55/LConn1
  _CN_352399506_110000_CN_103428598_110000/RConn1 -- T_103428598_220000;110000_/LConn1 -- _CN_136370548_110000_CN_103428598_110000/LConn1 -- _CN_103428598_110000_CN_104060546_110000/LConn1 -- _CN_103428598_110000_CN_150209972_110000/LConn1
  _CN_352399506_110000_CN_103428598_110000/RConn2 -- T_103428598_220000;110000_/LConn2 -- _CN_136370548_110000_CN_103428598_110000/LConn2 -- _CN_103428598_110000_CN_104060546_110000/LConn2 -- _CN_103428598_110000_CN_150209972_110000/LConn2
  _CN_352399506_110000_CN_103428598_110000/RConn3 -- T_103428598_220000;110000_/LConn3 -- _CN_136370548_110000_CN_103428598_110000/LConn3 -- _CN_103428598_110000_CN_104060546_110000/LConn3 -- _CN_103428598_110000_CN_150209972_110000/LConn3 -- bus56/LConn1
  _CN_25594007_110000_CN_28502182_110000/LConn1 -- T_25594007_400000;110000_Tammiston_sähköasema/RConn1 -- _CN_25594007_110000_CN_25597544_110000/LConn1 -- _CN_25594007_110000_CN_155555327_110000/LConn1 -- _CN_25594007_110000_CN_25598183_110000/LConn1 -- _CN_25594007_110000_CN_177308630_110000/LConn1 -- _CN_25594007_110000_CN_25593756_110000/LConn1 -- L_25594007/LConn1 -- _CN_25594007_110000_CN_31127270_110000/LConn1 -- _CN_25594007_110000_CN_28785740_110000/LConn1 -- _CN_25594007_110000_CN_26331359_110000/LConn1
  _CN_25594007_110000_CN_28502182_110000/LConn2 -- T_25594007_400000;110000_Tammiston_sähköasema/RConn2 -- _CN_25594007_110000_CN_25597544_110000/LConn2 -- _CN_25594007_110000_CN_155555327_110000/LConn2 -- _CN_25594007_110000_CN_25598183_110000/LConn2 -- _CN_25594007_110000_CN_177308630_110000/LConn2 -- _CN_25594007_110000_CN_25593756_110000/LConn2 -- L_25594007/LConn2 -- _CN_25594007_110000_CN_31127270_110000/LConn2 -- _CN_25594007_110000_CN_28785740_110000/LConn2 -- _CN_25594007_110000_CN_26331359_110000/LConn2
  _CN_25594007_110000_CN_28502182_110000/LConn3 -- T_25594007_400000;110000_Tammiston_sähköasema/RConn3 -- _CN_25594007_110000_CN_25597544_110000/LConn3 -- _CN_25594007_110000_CN_155555327_110000/LConn3 -- _CN_25594007_110000_CN_25598183_110000/LConn3 -- _CN_25594007_110000_CN_177308630_110000/LConn3 -- _CN_25594007_110000_CN_25593756_110000/LConn3 -- L_25594007/LConn3 -- bus57/LConn1 -- _CN_25594007_110000_CN_31127270_110000/LConn3 -- _CN_25594007_110000_CN_28785740_110000/LConn3 -- _CN_25594007_110000_CN_26331359_110000/LConn3
  _CN_25594007_110000_CN_28502182_110000/RConn1 -- T_28502182_110000_/LConn1 -- _CN_28502182_110000_CN_25598183_110000/LConn1
  _CN_25594007_110000_CN_28502182_110000/RConn2 -- T_28502182_110000_/LConn2 -- _CN_28502182_110000_CN_25598183_110000/LConn2
  _CN_25594007_110000_CN_28502182_110000/RConn3 -- T_28502182_110000_/LConn3 -- _CN_28502182_110000_CN_25598183_110000/LConn3 -- bus58/LConn1
  T_31127270_110000_/LConn1 -- _CN_25594007_110000_CN_31127270_110000/RConn1
  T_31127270_110000_/LConn2 -- _CN_25594007_110000_CN_31127270_110000/RConn2
  _CN_25594007_110000_CN_31127270_110000/RConn3 -- T_31127270_110000_/LConn3 -- bus59/LConn1
  _CN_25594007_110000_CN_28785740_110000/RConn1 -- T_28785740_110000_/LConn1 -- _CN_28785740_110000_CN_43140269_110000/LConn1 -- _CN_28785740_110000_CN_28820749_110000/LConn1
  _CN_25594007_110000_CN_28785740_110000/RConn2 -- T_28785740_110000_/LConn2 -- _CN_28785740_110000_CN_43140269_110000/LConn2 -- _CN_28785740_110000_CN_28820749_110000/LConn2
  _CN_25594007_110000_CN_28785740_110000/RConn3 -- T_28785740_110000_/LConn3 -- _CN_28785740_110000_CN_43140269_110000/LConn3 -- _CN_28785740_110000_CN_28820749_110000/LConn3 -- bus60/LConn1
  _CN_25594007_110000_CN_26331359_110000/RConn1 -- T_26331359_110000_/LConn1 -- _CN_26331359_110000_CN_43140269_110000/LConn1 -- _CN_26331359_110000_CN_6268760_110000/RConn1
  _CN_25594007_110000_CN_26331359_110000/RConn2 -- T_26331359_110000_/LConn2 -- _CN_26331359_110000_CN_43140269_110000/LConn2 -- _CN_26331359_110000_CN_6268760_110000/RConn2
  _CN_25594007_110000_CN_26331359_110000/RConn3 -- T_26331359_110000_/LConn3 -- _CN_26331359_110000_CN_43140269_110000/LConn3 -- bus61/LConn1 -- _CN_26331359_110000_CN_6268760_110000/RConn3
  T_25597544__Kannelmaki/LConn1 -- _CN_25594007_110000_CN_25597544_110000/RConn1
  T_25597544__Kannelmaki/LConn2 -- _CN_25594007_110000_CN_25597544_110000/RConn2
  _CN_25594007_110000_CN_25597544_110000/RConn3 -- T_25597544__Kannelmaki/LConn3 -- bus62/LConn1
  T_155555327_110000_Myyrmäen_sähköasema/LConn1 -- _CN_25594007_110000_CN_155555327_110000/RConn1
  T_155555327_110000_Myyrmäen_sähköasema/LConn2 -- _CN_25594007_110000_CN_155555327_110000/RConn2
  _CN_25594007_110000_CN_155555327_110000/RConn3 -- T_155555327_110000_Myyrmäen_sähköasema/LConn3 -- bus63/LConn1
  _CN_25594007_110000_CN_25598183_110000/RConn1 -- T_25598183__/LConn1 -- _CN_28502182_110000_CN_25598183_110000/RConn1 -- _CN_25598183_110000_CN_28085992_110000/LConn1
  _CN_25594007_110000_CN_25598183_110000/RConn2 -- T_25598183__/LConn2 -- _CN_28502182_110000_CN_25598183_110000/RConn2 -- _CN_25598183_110000_CN_28085992_110000/LConn2
  _CN_25594007_110000_CN_25598183_110000/RConn3 -- T_25598183__/LConn3 -- _CN_28502182_110000_CN_25598183_110000/RConn3 -- _CN_25598183_110000_CN_28085992_110000/LConn3 -- bus64/LConn1
  T_177308630_110000_/LConn1 -- _CN_25594007_110000_CN_177308630_110000/RConn1
  T_177308630_110000_/LConn2 -- _CN_25594007_110000_CN_177308630_110000/RConn2
  _CN_25594007_110000_CN_177308630_110000/RConn3 -- T_177308630_110000_/LConn3 -- bus65/LConn1
  _CN_25594007_110000_CN_25593756_110000/RConn1 -- T_25593756_110000_Viikki/LConn1 -- _CN_26391332_110000_CN_25593756_110000/LConn1
  _CN_25594007_110000_CN_25593756_110000/RConn2 -- T_25593756_110000_Viikki/LConn2 -- _CN_26391332_110000_CN_25593756_110000/LConn2
  _CN_25594007_110000_CN_25593756_110000/RConn3 -- T_25593756_110000_Viikki/LConn3 -- _CN_26391332_110000_CN_25593756_110000/LConn3 -- bus66/LConn1
  _CN_136363036_110000_CN_152333104_110000/LConn1 -- T_136363036_110000_/LConn1 -- _CN_136363036_110000_CN_130069838_110000/LConn1
  _CN_136363036_110000_CN_152333104_110000/LConn2 -- T_136363036_110000_/LConn2 -- _CN_136363036_110000_CN_130069838_110000/LConn2
  _CN_136363036_110000_CN_152333104_110000/LConn3 -- T_136363036_110000_/LConn3 -- _CN_136363036_110000_CN_130069838_110000/LConn3 -- bus67/LConn1
  _CN_136363036_110000_CN_152333104_110000/RConn1 -- T_152333104_110000_/LConn1 -- _CN_159693074_110000_CN_152333104_110000/LConn1
  _CN_136363036_110000_CN_152333104_110000/RConn2 -- T_152333104_110000_/LConn2 -- _CN_159693074_110000_CN_152333104_110000/LConn2
  _CN_136363036_110000_CN_152333104_110000/RConn3 -- T_152333104_110000_/LConn3 -- _CN_159693074_110000_CN_152333104_110000/LConn3 -- bus68/LConn1
  _CN_136363036_110000_CN_130069838_110000/RConn1 -- T_130069838__/LConn1 -- _CN_130069833_110000_CN_130069838_110000/LConn1
  _CN_136363036_110000_CN_130069838_110000/RConn2 -- T_130069838__/LConn2 -- _CN_130069833_110000_CN_130069838_110000/LConn2
  _CN_136363036_110000_CN_130069838_110000/RConn3 -- T_130069838__/LConn3 -- _CN_130069833_110000_CN_130069838_110000/LConn3 -- bus69/LConn1
  _CN_145567915_110000_CN_136909652_110000/LConn1 -- T_145567915_110000_/LConn1 -- _CN_145567915_110000_CN_136068907_110000/LConn1
  _CN_145567915_110000_CN_136909652_110000/LConn2 -- T_145567915_110000_/LConn2 -- _CN_145567915_110000_CN_136068907_110000/LConn2
  _CN_145567915_110000_CN_136909652_110000/LConn3 -- T_145567915_110000_/LConn3 -- _CN_145567915_110000_CN_136068907_110000/LConn3 -- bus70/LConn1
  T_136909652__/LConn1 -- _CN_145567915_110000_CN_136909652_110000/RConn1
  T_136909652__/LConn2 -- _CN_145567915_110000_CN_136909652_110000/RConn2
  _CN_145567915_110000_CN_136909652_110000/RConn3 -- T_136909652__/LConn3 -- bus71/LConn1
  _CN_145567915_110000_CN_136068907_110000/RConn1 -- T_136068907_400000;220000;110000_/RConn1 -- _CN_130069833_110000_CN_136068907_110000/LConn1 -- _CN_152740092_110000_CN_136068907_110000/LConn1 -- _CN_142434847_110000_CN_136068907_110000/LConn1
  _CN_145567915_110000_CN_136068907_110000/RConn2 -- T_136068907_400000;220000;110000_/RConn2 -- _CN_130069833_110000_CN_136068907_110000/LConn2 -- _CN_152740092_110000_CN_136068907_110000/LConn2 -- _CN_142434847_110000_CN_136068907_110000/LConn2
  _CN_145567915_110000_CN_136068907_110000/RConn3 -- T_136068907_400000;220000;110000_/RConn3 -- _CN_130069833_110000_CN_136068907_110000/LConn3 -- bus72/LConn1 -- _CN_152740092_110000_CN_136068907_110000/LConn3 -- _CN_142434847_110000_CN_136068907_110000/LConn3
  T_186886932_110000_/LConn1 -- _CN_43143343_110000_CN_186886932_110000/RConn1
  T_186886932_110000_/LConn2 -- _CN_43143343_110000_CN_186886932_110000/RConn2
  _CN_43143343_110000_CN_186886932_110000/RConn3 -- T_186886932_110000_/LConn3 -- bus73/LConn1
  _CN_43143343_110000_CN_128255187_110000/RConn1 -- T_128255187_110000_/LConn1 -- _CN_32910454_110000_CN_128255187_110000/LConn1
  _CN_43143343_110000_CN_128255187_110000/RConn2 -- T_128255187_110000_/LConn2 -- _CN_32910454_110000_CN_128255187_110000/LConn2
  _CN_43143343_110000_CN_128255187_110000/RConn3 -- T_128255187_110000_/LConn3 -- _CN_32910454_110000_CN_128255187_110000/LConn3 -- bus74/LConn1
  T_397651041__/LConn1 -- _CN_397651041_110000_CN_375670534_110000/LConn1
  T_397651041__/LConn2 -- _CN_397651041_110000_CN_375670534_110000/LConn2
  _CN_397651041_110000_CN_375670534_110000/LConn3 -- T_397651041__/LConn3 -- bus75/LConn1
  T_375670534_110000_/LConn1 -- _CN_397651041_110000_CN_375670534_110000/RConn1
  T_375670534_110000_/LConn2 -- _CN_397651041_110000_CN_375670534_110000/RConn2
  _CN_397651041_110000_CN_375670534_110000/RConn3 -- T_375670534_110000_/LConn3 -- bus76/LConn1
  T_169224396__Pyhäveden_sähköasema/LConn1 -- _CN_169224396_110000_CN_242586528_110000/LConn1
  T_169224396__Pyhäveden_sähköasema/LConn2 -- _CN_169224396_110000_CN_242586528_110000/LConn2
  _CN_169224396_110000_CN_242586528_110000/LConn3 -- T_169224396__Pyhäveden_sähköasema/LConn3 -- bus77/LConn1
  _CN_169224396_110000_CN_242586528_110000/RConn1 -- T_242586528_110000_/LConn1 -- _CN_140677655_110000_CN_242586528_110000/LConn1
  _CN_169224396_110000_CN_242586528_110000/RConn2 -- T_242586528_110000_/LConn2 -- _CN_140677655_110000_CN_242586528_110000/LConn2
  _CN_169224396_110000_CN_242586528_110000/RConn3 -- T_242586528_110000_/LConn3 -- _CN_140677655_110000_CN_242586528_110000/LConn3 -- bus78/LConn1
  _CN_26331359_110000_CN_43140269_110000/RConn1 -- T_43140269__Vuosaaren_sähköasema/LConn1 -- _CN_28785740_110000_CN_43140269_110000/RConn1
  _CN_26331359_110000_CN_43140269_110000/RConn2 -- T_43140269__Vuosaaren_sähköasema/LConn2 -- _CN_28785740_110000_CN_43140269_110000/RConn2
  _CN_26331359_110000_CN_43140269_110000/RConn3 -- T_43140269__Vuosaaren_sähköasema/LConn3 -- _CN_28785740_110000_CN_43140269_110000/RConn3 -- bus79/LConn1
  T_87697632__/LConn1 -- _CN_87697632_110000_CN_363802509_110000/LConn1
  T_87697632__/LConn2 -- _CN_87697632_110000_CN_363802509_110000/LConn2
  _CN_87697632_110000_CN_363802509_110000/LConn3 -- T_87697632__/LConn3 -- bus80/LConn1
  T_363802509_110000_/LConn1 -- _CN_87697632_110000_CN_363802509_110000/RConn1
  T_363802509_110000_/LConn2 -- _CN_87697632_110000_CN_363802509_110000/RConn2
  _CN_87697632_110000_CN_363802509_110000/RConn3 -- T_363802509_110000_/LConn3 -- bus81/LConn1
  _CN_238856422_110000_CN_219227505_110000/LConn1 -- T_238856422_400000;110000_/RConn1 -- L_238856422/LConn1
  _CN_238856422_110000_CN_219227505_110000/LConn2 -- T_238856422_400000;110000_/RConn2 -- L_238856422/LConn2
  _CN_238856422_110000_CN_219227505_110000/LConn3 -- T_238856422_400000;110000_/RConn3 -- L_238856422/LConn3 -- bus82/LConn1
  _CN_238856422_110000_CN_219227505_110000/RConn1 -- T_219227505__/LConn1 -- _CN_348003562_110000_CN_219227505_110000/LConn1
  _CN_238856422_110000_CN_219227505_110000/RConn2 -- T_219227505__/LConn2 -- _CN_348003562_110000_CN_219227505_110000/LConn2
  _CN_238856422_110000_CN_219227505_110000/RConn3 -- T_219227505__/LConn3 -- _CN_348003562_110000_CN_219227505_110000/LConn3 -- bus83/LConn1
  T_28085992__/LConn1 -- _CN_25598183_110000_CN_28085992_110000/RConn1
  T_28085992__/LConn2 -- _CN_25598183_110000_CN_28085992_110000/RConn2
  _CN_25598183_110000_CN_28085992_110000/RConn3 -- T_28085992__/LConn3 -- bus84/LConn1
  T_299874537__/LConn1 -- _CN_299874537_110000_CN_26501426_110000/LConn1
  T_299874537__/LConn2 -- _CN_299874537_110000_CN_26501426_110000/LConn2
  _CN_299874537_110000_CN_26501426_110000/LConn3 -- T_299874537__/LConn3 -- bus85/LConn1
  _CN_299874537_110000_CN_26501426_110000/RConn1 -- T_26501426_400000;110000_/RConn1 -- _CN_98576761_110000_CN_26501426_110000/LConn1 -- _CN_26501426_110000_CN_400582573_110000/LConn1 -- _CN_26501426_110000_CN_400582583_110000/LConn1 -- _CN_26501426_110000_CN_98613134_110000/LConn1 -- L_26501426/LConn1
  _CN_299874537_110000_CN_26501426_110000/RConn2 -- T_26501426_400000;110000_/RConn2 -- _CN_98576761_110000_CN_26501426_110000/LConn2 -- _CN_26501426_110000_CN_400582573_110000/LConn2 -- _CN_26501426_110000_CN_400582583_110000/LConn2 -- _CN_26501426_110000_CN_98613134_110000/LConn2 -- L_26501426/LConn2
  _CN_299874537_110000_CN_26501426_110000/RConn3 -- T_26501426_400000;110000_/RConn3 -- _CN_98576761_110000_CN_26501426_110000/LConn3 -- _CN_26501426_110000_CN_400582573_110000/LConn3 -- _CN_26501426_110000_CN_400582583_110000/LConn3 -- _CN_26501426_110000_CN_98613134_110000/LConn3 -- L_26501426/LConn3 -- bus86/LConn1
  T_143778041_110000_/LConn1 -- _CN_143778041_110000_CN_149954884_110000/LConn1
  T_143778041_110000_/LConn2 -- _CN_143778041_110000_CN_149954884_110000/LConn2
  _CN_143778041_110000_CN_149954884_110000/LConn3 -- T_143778041_110000_/LConn3 -- bus87/LConn1
  _CN_143778041_110000_CN_149954884_110000/RConn1 -- T_149954884_110000_/LConn1 -- _CN_149954884_110000_CN_98736918_110000/LConn1
  _CN_143778041_110000_CN_149954884_110000/RConn2 -- T_149954884_110000_/LConn2 -- _CN_149954884_110000_CN_98736918_110000/LConn2
  _CN_143778041_110000_CN_149954884_110000/RConn3 -- T_149954884_110000_/LConn3 -- _CN_149954884_110000_CN_98736918_110000/LConn3 -- bus88/LConn1
  _CN_152740092_110000_CN_149818658_110000/LConn1 -- T_152740092_110000_/LConn1 -- _CN_152740092_110000_CN_136068907_110000/RConn1
  _CN_152740092_110000_CN_149818658_110000/LConn2 -- T_152740092_110000_/LConn2 -- _CN_152740092_110000_CN_136068907_110000/RConn2
  _CN_152740092_110000_CN_149818658_110000/LConn3 -- T_152740092_110000_/LConn3 -- _CN_152740092_110000_CN_136068907_110000/RConn3 -- bus89/LConn1
  _CN_152740092_110000_CN_149818658_110000/RConn1 -- T_149818658_110000_/LConn1 -- _CN_149818658_110000_CN_149818659_110000/LConn1
  _CN_152740092_110000_CN_149818658_110000/RConn2 -- T_149818658_110000_/LConn2 -- _CN_149818658_110000_CN_149818659_110000/LConn2
  _CN_152740092_110000_CN_149818658_110000/RConn3 -- T_149818658_110000_/LConn3 -- _CN_149818658_110000_CN_149818659_110000/LConn3 -- bus90/LConn1
  T_159693074__/LConn1 -- _CN_159693074_110000_CN_152333104_110000/RConn1
  T_159693074__/LConn2 -- _CN_159693074_110000_CN_152333104_110000/RConn2
  _CN_159693074_110000_CN_152333104_110000/RConn3 -- T_159693074__/LConn3 -- bus91/LConn1
  T_152181013_110000_/LConn1 -- _CN_152181013_110000_CN_151818544_110000/LConn1
  T_152181013_110000_/LConn2 -- _CN_152181013_110000_CN_151818544_110000/LConn2
  _CN_152181013_110000_CN_151818544_110000/LConn3 -- T_152181013_110000_/LConn3 -- bus92/LConn1
  _CN_152181013_110000_CN_151818544_110000/RConn1 -- T_151818544_400000;110000_/RConn1 -- _CN_151818544_110000_CN_28017392_110000/LConn1 -- _CN_151818544_110000_CN_51420019_110000/LConn1 -- _CN_151818544_110000_CN_400588216_110000/LConn1 -- L_151818544/LConn1 -- _CN_151818544_110000_CN_400584163_110000/LConn1 -- _CN_151818544_110000_CN_151818564_110000/LConn1 -- _CN_151818544_110000_CN_168877874_110000/LConn1
  _CN_152181013_110000_CN_151818544_110000/RConn2 -- T_151818544_400000;110000_/RConn2 -- _CN_151818544_110000_CN_28017392_110000/LConn2 -- _CN_151818544_110000_CN_51420019_110000/LConn2 -- _CN_151818544_110000_CN_400588216_110000/LConn2 -- L_151818544/LConn2 -- _CN_151818544_110000_CN_400584163_110000/LConn2 -- _CN_151818544_110000_CN_151818564_110000/LConn2 -- _CN_151818544_110000_CN_168877874_110000/LConn2
  _CN_152181013_110000_CN_151818544_110000/RConn3 -- T_151818544_400000;110000_/RConn3 -- _CN_151818544_110000_CN_28017392_110000/LConn3 -- _CN_151818544_110000_CN_51420019_110000/LConn3 -- _CN_151818544_110000_CN_400588216_110000/LConn3 -- L_151818544/LConn3 -- bus93/LConn1 -- _CN_151818544_110000_CN_400584163_110000/LConn3 -- _CN_151818544_110000_CN_151818564_110000/LConn3 -- _CN_151818544_110000_CN_168877874_110000/LConn3
  _CN_157677847_110000_CN_302047780_110000/LConn1 -- T_157677847_110000_/LConn1 -- _CN_157677847_110000_CN_57845262_110000/LConn1
  _CN_157677847_110000_CN_302047780_110000/LConn2 -- T_157677847_110000_/LConn2 -- _CN_157677847_110000_CN_57845262_110000/LConn2
  _CN_157677847_110000_CN_302047780_110000/LConn3 -- T_157677847_110000_/LConn3 -- _CN_157677847_110000_CN_57845262_110000/LConn3 -- bus94/LConn1
  _CN_157677847_110000_CN_302047780_110000/RConn1 -- T_302047780_110000_/LConn1 -- _CN_302047780_110000_CN_88140424_110000/LConn1
  _CN_157677847_110000_CN_302047780_110000/RConn2 -- T_302047780_110000_/LConn2 -- _CN_302047780_110000_CN_88140424_110000/LConn2
  _CN_157677847_110000_CN_302047780_110000/RConn3 -- T_302047780_110000_/LConn3 -- _CN_302047780_110000_CN_88140424_110000/LConn3 -- bus95/LConn1
  _CN_157677847_110000_CN_57845262_110000/RConn1 -- T_57845262_110000_/LConn1 -- Tuovila_Vaskiluoto_CN_93624966_110000_CN_57845262_110000/LConn1
  _CN_157677847_110000_CN_57845262_110000/RConn2 -- T_57845262_110000_/LConn2 -- Tuovila_Vaskiluoto_CN_93624966_110000_CN_57845262_110000/LConn2
  _CN_157677847_110000_CN_57845262_110000/RConn3 -- T_57845262_110000_/LConn3 -- Tuovila_Vaskiluoto_CN_93624966_110000_CN_57845262_110000/LConn3 -- bus96/LConn1
  T_119141766__/LConn1 -- _CN_119141766_110000_CN_34623113_110000/LConn1
  T_119141766__/LConn2 -- _CN_119141766_110000_CN_34623113_110000/LConn2
  _CN_119141766_110000_CN_34623113_110000/LConn3 -- T_119141766__/LConn3 -- bus97/LConn1
  _CN_119141766_110000_CN_34623113_110000/RConn1 -- T_34623113_400000;110000_/RConn1 -- _CN_152315970_110000_CN_34623113_110000/LConn1 -- L_34623113/LConn1
  _CN_119141766_110000_CN_34623113_110000/RConn2 -- T_34623113_400000;110000_/RConn2 -- _CN_152315970_110000_CN_34623113_110000/LConn2 -- L_34623113/LConn2
  _CN_119141766_110000_CN_34623113_110000/RConn3 -- T_34623113_400000;110000_/RConn3 -- _CN_152315970_110000_CN_34623113_110000/LConn3 -- L_34623113/LConn3 -- bus98/LConn1
  T_399014185_110000_/LConn1 -- _CN_399014185_110000_CN_379937972_110000/LConn1
  T_399014185_110000_/LConn2 -- _CN_399014185_110000_CN_379937972_110000/LConn2
  _CN_399014185_110000_CN_379937972_110000/LConn3 -- T_399014185_110000_/LConn3 -- bus99/LConn1
  T_379937972_220000_/LConn1 -- _CN_399014185_110000_CN_379937972_110000/RConn1
  T_379937972_220000_/LConn2 -- _CN_399014185_110000_CN_379937972_110000/RConn2
  _CN_399014185_110000_CN_379937972_110000/RConn3 -- T_379937972_220000_/LConn3 -- bus100/LConn1
  T_168877874_110000_/LConn1 -- _CN_151818544_110000_CN_168877874_110000/RConn1
  T_168877874_110000_/LConn2 -- _CN_151818544_110000_CN_168877874_110000/RConn2
  _CN_151818544_110000_CN_168877874_110000/RConn3 -- T_168877874_110000_/LConn3 -- bus101/LConn1
  _CN_151818544_110000_CN_400584163_110000/RConn1 -- T_400584163__/LConn1 -- _CN_98735006_110000_CN_400584163_110000/LConn1 -- _CN_151818569_110000_CN_400584163_110000/LConn1
  _CN_151818544_110000_CN_400584163_110000/RConn2 -- T_400584163__/LConn2 -- _CN_98735006_110000_CN_400584163_110000/LConn2 -- _CN_151818569_110000_CN_400584163_110000/LConn2
  _CN_151818544_110000_CN_400584163_110000/RConn3 -- T_400584163__/LConn3 -- _CN_98735006_110000_CN_400584163_110000/LConn3 -- bus102/LConn1 -- _CN_151818569_110000_CN_400584163_110000/LConn3
  T_151818564_110000_/LConn1 -- _CN_151818544_110000_CN_151818564_110000/RConn1
  T_151818564_110000_/LConn2 -- _CN_151818544_110000_CN_151818564_110000/RConn2
  _CN_151818544_110000_CN_151818564_110000/RConn3 -- T_151818564_110000_/LConn3 -- bus103/LConn1
  G_28017392_Koroisten_sähköasema/RConn1 -- _CN_151818544_110000_CN_28017392_110000/RConn1
  G_28017392_Koroisten_sähköasema/RConn2 -- _CN_151818544_110000_CN_28017392_110000/RConn2
  _CN_151818544_110000_CN_28017392_110000/RConn3 -- G_28017392_Koroisten_sähköasema/RConn3 -- bus104/LConn1
  T_51420019_110000_/LConn1 -- _CN_151818544_110000_CN_51420019_110000/RConn1
  T_51420019_110000_/LConn2 -- _CN_151818544_110000_CN_51420019_110000/RConn2
  _CN_151818544_110000_CN_51420019_110000/RConn3 -- T_51420019_110000_/LConn3 -- bus105/LConn1
  _CN_151818544_110000_CN_400588216_110000/RConn1 -- T_400588216_110000_/LConn1 -- _CN_400588215_110000_CN_400588216_110000/LConn1
  _CN_151818544_110000_CN_400588216_110000/RConn2 -- T_400588216_110000_/LConn2 -- _CN_400588215_110000_CN_400588216_110000/LConn2
  _CN_151818544_110000_CN_400588216_110000/RConn3 -- T_400588216_110000_/LConn3 -- _CN_400588215_110000_CN_400588216_110000/LConn3 -- bus106/LConn1
  T_143419698_110000;25000_Lamminpää_SA/LConn1 -- _CN_143419698_110000_CN_142846914_110000/LConn1
  T_143419698_110000;25000_Lamminpää_SA/LConn2 -- _CN_143419698_110000_CN_142846914_110000/LConn2
  _CN_143419698_110000_CN_142846914_110000/LConn3 -- T_143419698_110000;25000_Lamminpää_SA/LConn3 -- bus107/LConn1
  T_142846914_110000_/LConn1 -- _CN_143419698_110000_CN_142846914_110000/RConn1
  T_142846914_110000_/LConn2 -- _CN_143419698_110000_CN_142846914_110000/RConn2
  _CN_143419698_110000_CN_142846914_110000/RConn3 -- T_142846914_110000_/LConn3 -- bus108/LConn1
  _CN_161022271_110000_CN_161022023_110000/LConn1 -- T_161022271_110000_/LConn1 -- _CN_161022271_110000_CN_154863454_110000/LConn1
  _CN_161022271_110000_CN_161022023_110000/LConn2 -- T_161022271_110000_/LConn2 -- _CN_161022271_110000_CN_154863454_110000/LConn2
  _CN_161022271_110000_CN_161022023_110000/LConn3 -- T_161022271_110000_/LConn3 -- _CN_161022271_110000_CN_154863454_110000/LConn3 -- bus109/LConn1
  _CN_161022271_110000_CN_161022023_110000/RConn1 -- T_161022023__/LConn1 -- _CN_161022023_110000_CN_142035550_110000/LConn1 -- _CN_161022023_110000_CN_35281467_110000/LConn1
  _CN_161022271_110000_CN_161022023_110000/RConn2 -- T_161022023__/LConn2 -- _CN_161022023_110000_CN_142035550_110000/LConn2 -- _CN_161022023_110000_CN_35281467_110000/LConn2
  _CN_161022271_110000_CN_161022023_110000/RConn3 -- T_161022023__/LConn3 -- _CN_161022023_110000_CN_142035550_110000/LConn3 -- bus110/LConn1 -- _CN_161022023_110000_CN_35281467_110000/LConn3
  _CN_161022271_110000_CN_154863454_110000/RConn1 -- T_154863454_110000_/LConn1 -- _CN_165373253_110000_CN_154863454_110000/LConn1
  _CN_161022271_110000_CN_154863454_110000/RConn2 -- T_154863454_110000_/LConn2 -- _CN_165373253_110000_CN_154863454_110000/LConn2
  _CN_161022271_110000_CN_154863454_110000/RConn3 -- T_154863454_110000_/LConn3 -- _CN_165373253_110000_CN_154863454_110000/LConn3 -- bus111/LConn1
  _CN_149954884_110000_CN_98736918_110000/RConn1 -- T_98736918_400000;110000_/RConn1 -- _CN_98736918_110000_CN_158031219_110000/LConn1 -- L_98736918/LConn1 -- _CN_158104293_110000_CN_98736918_110000/LConn1
  _CN_149954884_110000_CN_98736918_110000/RConn2 -- T_98736918_400000;110000_/RConn2 -- _CN_98736918_110000_CN_158031219_110000/LConn2 -- L_98736918/LConn2 -- _CN_158104293_110000_CN_98736918_110000/LConn2
  _CN_149954884_110000_CN_98736918_110000/RConn3 -- T_98736918_400000;110000_/RConn3 -- _CN_98736918_110000_CN_158031219_110000/LConn3 -- L_98736918/LConn3 -- bus112/LConn1 -- _CN_158104293_110000_CN_98736918_110000/LConn3
  T_151818569_110000_/LConn1 -- _CN_151818569_110000_CN_400584163_110000/RConn1
  T_151818569_110000_/LConn2 -- _CN_151818569_110000_CN_400584163_110000/RConn2
  _CN_151818569_110000_CN_400584163_110000/RConn3 -- T_151818569_110000_/LConn3 -- bus113/LConn1
  _CN_320110941_110000_CN_151206413_110000/LConn1 -- T_320110941_110000;25000_Rännäri_SA/LConn1 -- _CN_320110941_110000_CN_142846913_110000/LConn1
  _CN_320110941_110000_CN_151206413_110000/LConn2 -- T_320110941_110000;25000_Rännäri_SA/LConn2 -- _CN_320110941_110000_CN_142846913_110000/LConn2
  _CN_320110941_110000_CN_151206413_110000/LConn3 -- T_320110941_110000;25000_Rännäri_SA/LConn3 -- _CN_320110941_110000_CN_142846913_110000/LConn3 -- bus114/LConn1
  _CN_320110941_110000_CN_151206413_110000/RConn1 -- T_151206413_110000;25000_Pahaneva_SA/LConn1 -- _CN_151206413_110000_CN_168049346_110000/LConn1
  _CN_320110941_110000_CN_151206413_110000/RConn2 -- T_151206413_110000;25000_Pahaneva_SA/LConn2 -- _CN_151206413_110000_CN_168049346_110000/LConn2
  _CN_320110941_110000_CN_151206413_110000/RConn3 -- T_151206413_110000;25000_Pahaneva_SA/LConn3 -- _CN_151206413_110000_CN_168049346_110000/LConn3 -- bus115/LConn1
  _CN_320110941_110000_CN_142846913_110000/RConn1 -- T_142846913_110000;25000_Sisättö_SA/LConn1 -- _CN_142846911_110000_CN_142846913_110000/LConn1
  _CN_320110941_110000_CN_142846913_110000/RConn2 -- T_142846913_110000;25000_Sisättö_SA/LConn2 -- _CN_142846911_110000_CN_142846913_110000/LConn2
  _CN_320110941_110000_CN_142846913_110000/RConn3 -- T_142846913_110000;25000_Sisättö_SA/LConn3 -- _CN_142846911_110000_CN_142846913_110000/LConn3 -- bus116/LConn1
  T_159825638_110000_/LConn1 -- _CN_159825638_110000_CN_140834620_110000/LConn1
  T_159825638_110000_/LConn2 -- _CN_159825638_110000_CN_140834620_110000/LConn2
  _CN_159825638_110000_CN_140834620_110000/LConn3 -- T_159825638_110000_/LConn3 -- bus117/LConn1
  _CN_159825638_110000_CN_140834620_110000/RConn1 -- T_140834620_110000_/LConn1 -- _CN_140677655_110000_CN_140834620_110000/LConn1
  _CN_159825638_110000_CN_140834620_110000/RConn2 -- T_140834620_110000_/LConn2 -- _CN_140677655_110000_CN_140834620_110000/LConn2
  _CN_159825638_110000_CN_140834620_110000/RConn3 -- T_140834620_110000_/LConn3 -- _CN_140677655_110000_CN_140834620_110000/LConn3 -- bus118/LConn1
  _CN_200407399_110000_CN_26329645_110000/LConn1 -- T_200407399__/LConn1 -- _CN_200407399_110000_CN_128463750_110000/LConn1
  _CN_200407399_110000_CN_26329645_110000/LConn2 -- T_200407399__/LConn2 -- _CN_200407399_110000_CN_128463750_110000/LConn2
  _CN_200407399_110000_CN_26329645_110000/LConn3 -- T_200407399__/LConn3 -- _CN_200407399_110000_CN_128463750_110000/LConn3 -- bus119/LConn1
  T_26329645_110000_/LConn1 -- _CN_200407399_110000_CN_26329645_110000/RConn1
  T_26329645_110000_/LConn2 -- _CN_200407399_110000_CN_26329645_110000/RConn2
  _CN_200407399_110000_CN_26329645_110000/RConn3 -- T_26329645_110000_/LConn3 -- bus120/LConn1
  _CN_200407399_110000_CN_128463750_110000/RConn1 -- T_128463750_400000;110000_/RConn1 -- _CN_153187093_110000_CN_128463750_110000/LConn1 -- _CN_128463750_110000_CN_129112047_110000/LConn1 -- _CN_128463750_110000_CN_155899286_110000/LConn1 -- L_128463750/LConn1 -- _CN_151583286_110000_CN_128463750_110000/LConn1
  _CN_200407399_110000_CN_128463750_110000/RConn2 -- T_128463750_400000;110000_/RConn2 -- _CN_153187093_110000_CN_128463750_110000/LConn2 -- _CN_128463750_110000_CN_129112047_110000/LConn2 -- _CN_128463750_110000_CN_155899286_110000/LConn2 -- L_128463750/LConn2 -- _CN_151583286_110000_CN_128463750_110000/LConn2
  _CN_200407399_110000_CN_128463750_110000/RConn3 -- T_128463750_400000;110000_/RConn3 -- _CN_153187093_110000_CN_128463750_110000/LConn3 -- _CN_128463750_110000_CN_129112047_110000/LConn3 -- _CN_128463750_110000_CN_155899286_110000/LConn3 -- L_128463750/LConn3 -- bus121/LConn1 -- _CN_151583286_110000_CN_128463750_110000/LConn3
  T_259365224__/LConn1 -- _CN_259365224_110000_CN_158104301_110000/LConn1
  T_259365224__/LConn2 -- _CN_259365224_110000_CN_158104301_110000/LConn2
  _CN_259365224_110000_CN_158104301_110000/LConn3 -- T_259365224__/LConn3 -- bus122/LConn1
  T_158104301_110000_/LConn1 -- _CN_259365224_110000_CN_158104301_110000/RConn1
  T_158104301_110000_/LConn2 -- _CN_259365224_110000_CN_158104301_110000/RConn2
  _CN_259365224_110000_CN_158104301_110000/RConn3 -- T_158104301_110000_/LConn3 -- bus123/LConn1
  T_148312425__/LConn1 -- _CN_148312425_110000_CN_128571463_110000/RConn1
  T_148312425__/LConn2 -- _CN_148312425_110000_CN_128571463_110000/RConn2
  _CN_148312425_110000_CN_128571463_110000/RConn3 -- T_148312425__/LConn3 -- bus124/LConn1
  _CN_119130475_110000_CN_117383986_110000/LConn1 -- T_119130475_220000;110000_/LConn1 -- _CN_119130475_110000_CN_355823297_110000/LConn1
  _CN_119130475_110000_CN_117383986_110000/LConn2 -- T_119130475_220000;110000_/LConn2 -- _CN_119130475_110000_CN_355823297_110000/LConn2
  _CN_119130475_110000_CN_117383986_110000/LConn3 -- T_119130475_220000;110000_/LConn3 -- _CN_119130475_110000_CN_355823297_110000/LConn3 -- bus125/LConn1
  _CN_119130475_110000_CN_117383986_110000/RConn1 -- T_117383986_110000_/LConn1 -- _CN_117383986_110000_CN_153576520_110000/LConn1
  _CN_119130475_110000_CN_117383986_110000/RConn2 -- T_117383986_110000_/LConn2 -- _CN_117383986_110000_CN_153576520_110000/LConn2
  _CN_119130475_110000_CN_117383986_110000/RConn3 -- T_117383986_110000_/LConn3 -- _CN_117383986_110000_CN_153576520_110000/LConn3 -- bus126/LConn1
  T_355823297__/LConn1 -- _CN_119130475_110000_CN_355823297_110000/RConn1
  T_355823297__/LConn2 -- _CN_119130475_110000_CN_355823297_110000/RConn2
  _CN_119130475_110000_CN_355823297_110000/RConn3 -- T_355823297__/LConn3 -- bus127/LConn1
  T_192143731_110000_/LConn1 -- _CN_192143731_110000_CN_238900636_110000/LConn1
  T_192143731_110000_/LConn2 -- _CN_192143731_110000_CN_238900636_110000/LConn2
  _CN_192143731_110000_CN_238900636_110000/LConn3 -- T_192143731_110000_/LConn3 -- bus128/LConn1
  _CN_192143731_110000_CN_238900636_110000/RConn1 -- G_238900636_Inkoon_voimalaitos/RConn1 -- _CN_348003562_110000_CN_238900636_110000/LConn1 -- _CN_348003562_400000_CN_238900636_110000/LConn1
  _CN_192143731_110000_CN_238900636_110000/RConn2 -- G_238900636_Inkoon_voimalaitos/RConn2 -- _CN_348003562_110000_CN_238900636_110000/LConn2 -- _CN_348003562_400000_CN_238900636_110000/LConn2
  _CN_192143731_110000_CN_238900636_110000/RConn3 -- G_238900636_Inkoon_voimalaitos/RConn3 -- _CN_348003562_110000_CN_238900636_110000/LConn3 -- _CN_348003562_400000_CN_238900636_110000/LConn3 -- bus129/LConn1
  _CN_136370548_110000_CN_162675317_110000/LConn1 -- T_136370548_110000_/LConn1 -- _CN_136370548_110000_CN_148596527_110000/LConn1 -- _CN_136370548_110000_CN_103428598_110000/RConn1
  _CN_136370548_110000_CN_162675317_110000/LConn2 -- T_136370548_110000_/LConn2 -- _CN_136370548_110000_CN_148596527_110000/LConn2 -- _CN_136370548_110000_CN_103428598_110000/RConn2
  _CN_136370548_110000_CN_162675317_110000/LConn3 -- T_136370548_110000_/LConn3 -- _CN_136370548_110000_CN_148596527_110000/LConn3 -- _CN_136370548_110000_CN_103428598_110000/RConn3 -- bus130/LConn1
  T_162675317__/LConn1 -- _CN_136370548_110000_CN_162675317_110000/RConn1
  T_162675317__/LConn2 -- _CN_136370548_110000_CN_162675317_110000/RConn2
  _CN_136370548_110000_CN_162675317_110000/RConn3 -- T_162675317__/LConn3 -- bus131/LConn1
  _CN_136370548_110000_CN_148596527_110000/RConn1 -- T_148596527_110000_/LConn1 -- _CN_153576520_110000_CN_148596527_110000/LConn1
  _CN_136370548_110000_CN_148596527_110000/RConn2 -- T_148596527_110000_/LConn2 -- _CN_153576520_110000_CN_148596527_110000/LConn2
  _CN_136370548_110000_CN_148596527_110000/RConn3 -- T_148596527_110000_/LConn3 -- _CN_153576520_110000_CN_148596527_110000/LConn3 -- bus132/LConn1
  T_98576761_110000_/LConn1 -- _CN_98576761_110000_CN_26501426_110000/RConn1
  T_98576761_110000_/LConn2 -- _CN_98576761_110000_CN_26501426_110000/RConn2
  _CN_98576761_110000_CN_26501426_110000/RConn3 -- T_98576761_110000_/LConn3 -- bus133/LConn1
  T_217032427__/LConn1 -- _CN_217032427_110000_CN_118766661_110000/LConn1
  T_217032427__/LConn2 -- _CN_217032427_110000_CN_118766661_110000/LConn2
  _CN_217032427_110000_CN_118766661_110000/LConn3 -- T_217032427__/LConn3 -- bus134/LConn1
  _CN_217032427_110000_CN_118766661_110000/RConn1 -- T_118766661_110000_/LConn1 -- _CN_47317827_110000_CN_118766661_110000/LConn1
  _CN_217032427_110000_CN_118766661_110000/RConn2 -- T_118766661_110000_/LConn2 -- _CN_47317827_110000_CN_118766661_110000/LConn2
  _CN_217032427_110000_CN_118766661_110000/RConn3 -- T_118766661_110000_/LConn3 -- _CN_47317827_110000_CN_118766661_110000/LConn3 -- bus135/LConn1
  T_152315970_110000_/LConn1 -- _CN_152315970_110000_CN_34623113_110000/RConn1
  T_152315970_110000_/LConn2 -- _CN_152315970_110000_CN_34623113_110000/RConn2
  _CN_152315970_110000_CN_34623113_110000/RConn3 -- T_152315970_110000_/LConn3 -- bus136/LConn1
  T_97264036__/LConn1 -- _CN_97264036_110000_CN_40101584_110000/LConn1
  T_97264036__/LConn2 -- _CN_97264036_110000_CN_40101584_110000/LConn2
  _CN_97264036_110000_CN_40101584_110000/LConn3 -- T_97264036__/LConn3 -- bus137/LConn1
  _CN_97264036_110000_CN_40101584_110000/RConn1 -- T_40101584_110000_/LConn1 -- _CN_345672928_110000_CN_40101584_110000/LConn1 -- _CN_348349188_110000_CN_40101584_110000/LConn1 -- _CN_30483473_110000_CN_40101584_110000/LConn1
  _CN_97264036_110000_CN_40101584_110000/RConn2 -- T_40101584_110000_/LConn2 -- _CN_345672928_110000_CN_40101584_110000/LConn2 -- _CN_348349188_110000_CN_40101584_110000/LConn2 -- _CN_30483473_110000_CN_40101584_110000/LConn2
  _CN_97264036_110000_CN_40101584_110000/RConn3 -- T_40101584_110000_/LConn3 -- _CN_345672928_110000_CN_40101584_110000/LConn3 -- bus138/LConn1 -- _CN_348349188_110000_CN_40101584_110000/LConn3 -- _CN_30483473_110000_CN_40101584_110000/LConn3
  _CN_161022023_110000_CN_35281467_110000/RConn1 -- T_35281467_400000;110000_Korian_sähköasema/RConn1 -- _CN_35281467_110000_CN_178639425_110000/LConn1 -- L_35281467/LConn1 -- KR_KM_CN_166909843_110000_CN_35281467_110000/LConn1 -- _CN_140677655_110000_CN_35281467_110000/LConn1 -- _CN_35281467_110000_CN_167455825_110000/LConn1 -- _CN_35281467_110000_CN_348251886_110000/LConn1
  _CN_161022023_110000_CN_35281467_110000/RConn2 -- T_35281467_400000;110000_Korian_sähköasema/RConn2 -- _CN_35281467_110000_CN_178639425_110000/LConn2 -- L_35281467/LConn2 -- KR_KM_CN_166909843_110000_CN_35281467_110000/LConn2 -- _CN_140677655_110000_CN_35281467_110000/LConn2 -- _CN_35281467_110000_CN_167455825_110000/LConn2 -- _CN_35281467_110000_CN_348251886_110000/LConn2
  _CN_161022023_110000_CN_35281467_110000/RConn3 -- T_35281467_400000;110000_Korian_sähköasema/RConn3 -- _CN_35281467_110000_CN_178639425_110000/LConn3 -- L_35281467/LConn3 -- bus139/LConn1 -- KR_KM_CN_166909843_110000_CN_35281467_110000/LConn3 -- _CN_140677655_110000_CN_35281467_110000/LConn3 -- _CN_35281467_110000_CN_167455825_110000/LConn3 -- _CN_35281467_110000_CN_348251886_110000/LConn3
  _CN_161022023_110000_CN_142035550_110000/RConn1 -- T_142035550_110000_/LConn1 -- _CN_142035550_110000_CN_98561229_110000/LConn1
  _CN_161022023_110000_CN_142035550_110000/RConn2 -- T_142035550_110000_/LConn2 -- _CN_142035550_110000_CN_98561229_110000/LConn2
  _CN_161022023_110000_CN_142035550_110000/RConn3 -- T_142035550_110000_/LConn3 -- _CN_142035550_110000_CN_98561229_110000/LConn3 -- bus140/LConn1
  T_182503916_110000_/LConn1 -- _CN_182503916_110000_CN_364224532_110000/LConn1
  T_182503916_110000_/LConn2 -- _CN_182503916_110000_CN_364224532_110000/LConn2
  _CN_182503916_110000_CN_364224532_110000/LConn3 -- T_182503916_110000_/LConn3 -- bus141/LConn1
  T_364224532__/LConn1 -- _CN_182503916_110000_CN_364224532_110000/RConn1
  T_364224532__/LConn2 -- _CN_182503916_110000_CN_364224532_110000/RConn2
  _CN_182503916_110000_CN_364224532_110000/RConn3 -- T_364224532__/LConn3 -- bus142/LConn1
  T_104060546_110000_/LConn1 -- _CN_103428598_110000_CN_104060546_110000/RConn1
  T_104060546_110000_/LConn2 -- _CN_103428598_110000_CN_104060546_110000/RConn2
  _CN_103428598_110000_CN_104060546_110000/RConn3 -- T_104060546_110000_/LConn3 -- bus143/LConn1
  _CN_103428598_110000_CN_150209972_110000/RConn1 -- T_150209972_400000;110000_Tuovila/RConn1 -- _CN_168049346_110000_CN_150209972_110000/LConn1 -- Tuovila_Vaskiluoto_CN_93624966_110000_CN_150209972_110000/LConn1
  _CN_103428598_110000_CN_150209972_110000/RConn2 -- T_150209972_400000;110000_Tuovila/RConn2 -- _CN_168049346_110000_CN_150209972_110000/LConn2 -- Tuovila_Vaskiluoto_CN_93624966_110000_CN_150209972_110000/LConn2
  _CN_103428598_110000_CN_150209972_110000/RConn3 -- T_150209972_400000;110000_Tuovila/RConn3 -- _CN_168049346_110000_CN_150209972_110000/LConn3 -- bus144/LConn1 -- Tuovila_Vaskiluoto_CN_93624966_110000_CN_150209972_110000/LConn3
  T_166909843_110000_/LConn1 -- KR_KM_CN_166909843_110000_CN_35281467_110000/RConn1
  T_166909843_110000_/LConn2 -- KR_KM_CN_166909843_110000_CN_35281467_110000/RConn2
  KR_KM_CN_166909843_110000_CN_35281467_110000/RConn3 -- T_166909843_110000_/LConn3 -- bus145/LConn1
  T_377338368_110000_/LConn1 -- _CN_377338368_110000_CN_32910454_110000/LConn1
  T_377338368_110000_/LConn2 -- _CN_377338368_110000_CN_32910454_110000/LConn2
  _CN_377338368_110000_CN_32910454_110000/LConn3 -- T_377338368_110000_/LConn3 -- bus146/LConn1
  _CN_377338368_110000_CN_32910454_110000/RConn1 -- T_32910454__/LConn1 -- _CN_32910454_110000_CN_128255187_110000/RConn1 -- _CN_32910454_110000_CN_167705754_110000/LConn1 -- _CN_59014204_110000_CN_32910454_110000/RConn1 -- _CN_32910454_110000_CN_218734234_110000/LConn1
  _CN_377338368_110000_CN_32910454_110000/RConn2 -- T_32910454__/LConn2 -- _CN_32910454_110000_CN_128255187_110000/RConn2 -- _CN_32910454_110000_CN_167705754_110000/LConn2 -- _CN_59014204_110000_CN_32910454_110000/RConn2 -- _CN_32910454_110000_CN_218734234_110000/LConn2
  _CN_377338368_110000_CN_32910454_110000/RConn3 -- T_32910454__/LConn3 -- _CN_32910454_110000_CN_128255187_110000/RConn3 -- _CN_32910454_110000_CN_167705754_110000/LConn3 -- bus147/LConn1 -- _CN_59014204_110000_CN_32910454_110000/RConn3 -- _CN_32910454_110000_CN_218734234_110000/LConn3
  _CN_151206413_110000_CN_168049346_110000/RConn1 -- T_168049346_110000_Empower/LConn1 -- _CN_168049346_110000_CN_167040166_110000/LConn1 -- _CN_168049346_110000_CN_150209972_110000/RConn1 -- _CN_168049346_110000_CN_123462491_110000/LConn1
  _CN_151206413_110000_CN_168049346_110000/RConn2 -- T_168049346_110000_Empower/LConn2 -- _CN_168049346_110000_CN_167040166_110000/LConn2 -- _CN_168049346_110000_CN_150209972_110000/RConn2 -- _CN_168049346_110000_CN_123462491_110000/LConn2
  _CN_151206413_110000_CN_168049346_110000/RConn3 -- T_168049346_110000_Empower/LConn3 -- _CN_168049346_110000_CN_167040166_110000/LConn3 -- bus148/LConn1 -- _CN_168049346_110000_CN_150209972_110000/RConn3 -- _CN_168049346_110000_CN_123462491_110000/LConn3
  _CN_140677655_110000_CN_242586528_110000/RConn1 -- T_140677655_110000_/LConn1 -- _CN_140677655_110000_CN_35281467_110000/RConn1 -- _CN_140677655_110000_CN_140834620_110000/RConn1
  _CN_140677655_110000_CN_242586528_110000/RConn2 -- T_140677655_110000_/LConn2 -- _CN_140677655_110000_CN_35281467_110000/RConn2 -- _CN_140677655_110000_CN_140834620_110000/RConn2
  _CN_140677655_110000_CN_242586528_110000/RConn3 -- T_140677655_110000_/LConn3 -- _CN_140677655_110000_CN_35281467_110000/RConn3 -- _CN_140677655_110000_CN_140834620_110000/RConn3 -- bus149/LConn1
  T_363178756_220000;110000_/LConn1 -- _CN_363178756_110000_CN_205715364_110000/LConn1
  T_363178756_220000;110000_/LConn2 -- _CN_363178756_110000_CN_205715364_110000/LConn2
  _CN_363178756_110000_CN_205715364_110000/LConn3 -- T_363178756_220000;110000_/LConn3 -- bus150/LConn1
  _CN_363178756_110000_CN_205715364_110000/RConn1 -- T_205715364_110000_/LConn1 -- _CN_220230343_110000_CN_205715364_110000/LConn1
  _CN_363178756_110000_CN_205715364_110000/RConn2 -- T_205715364_110000_/LConn2 -- _CN_220230343_110000_CN_205715364_110000/LConn2
  _CN_363178756_110000_CN_205715364_110000/RConn3 -- T_205715364_110000_/LConn3 -- _CN_220230343_110000_CN_205715364_110000/LConn3 -- bus151/LConn1
  T_142434847_110000_/LConn1 -- _CN_142434847_110000_CN_136068907_110000/RConn1
  T_142434847_110000_/LConn2 -- _CN_142434847_110000_CN_136068907_110000/RConn2
  _CN_142434847_110000_CN_136068907_110000/RConn3 -- T_142434847_110000_/LConn3 -- bus152/LConn1
  G_88140424_Vaskiluodon_Voima_Oy/RConn1 -- _CN_302047780_110000_CN_88140424_110000/RConn1
  G_88140424_Vaskiluodon_Voima_Oy/RConn2 -- _CN_302047780_110000_CN_88140424_110000/RConn2
  _CN_302047780_110000_CN_88140424_110000/RConn3 -- G_88140424_Vaskiluodon_Voima_Oy/RConn3 -- bus153/LConn1
  T_255787563_110000_/LConn1 -- _CN_255787563_110000_CN_167186210_110000/LConn1
  T_255787563_110000_/LConn2 -- _CN_255787563_110000_CN_167186210_110000/LConn2
  _CN_255787563_110000_CN_167186210_110000/LConn3 -- T_255787563_110000_/LConn3 -- bus154/LConn1
  T_167186210_110000_/LConn1 -- _CN_255787563_110000_CN_167186210_110000/RConn1
  T_167186210_110000_/LConn2 -- _CN_255787563_110000_CN_167186210_110000/RConn2
  _CN_255787563_110000_CN_167186210_110000/RConn3 -- T_167186210_110000_/LConn3 -- bus155/LConn1
  _CN_151583286_110000_CN_128463750_110000/RConn1 -- T_151583286_110000_/LConn1 -- _CN_151583286_110000_CN_208979069_110000/RConn1
  _CN_151583286_110000_CN_128463750_110000/RConn2 -- T_151583286_110000_/LConn2 -- _CN_151583286_110000_CN_208979069_110000/RConn2
  _CN_151583286_110000_CN_128463750_110000/RConn3 -- T_151583286_110000_/LConn3 -- _CN_151583286_110000_CN_208979069_110000/RConn3 -- bus156/LConn1
  _CN_178307639_110000_CN_26619335_110000/LConn1 -- T_178307639__/LConn1 -- _CN_178307639_110000_CN_108980081_110000/RConn1
  _CN_178307639_110000_CN_26619335_110000/LConn2 -- T_178307639__/LConn2 -- _CN_178307639_110000_CN_108980081_110000/RConn2
  _CN_178307639_110000_CN_26619335_110000/LConn3 -- T_178307639__/LConn3 -- _CN_178307639_110000_CN_108980081_110000/RConn3 -- bus157/LConn1
  _CN_178307639_110000_CN_26619335_110000/RConn1 -- T_26619335_400000;110000_/RConn1 -- _CN_26619335_110000_CN_178234889_110000/LConn1 -- _CN_26619335_110000_CN_178234890_110000/LConn1 -- L_26619335/LConn1
  _CN_178307639_110000_CN_26619335_110000/RConn2 -- T_26619335_400000;110000_/RConn2 -- _CN_26619335_110000_CN_178234889_110000/LConn2 -- _CN_26619335_110000_CN_178234890_110000/LConn2 -- L_26619335/LConn2
  _CN_178307639_110000_CN_26619335_110000/RConn3 -- T_26619335_400000;110000_/RConn3 -- _CN_26619335_110000_CN_178234889_110000/LConn3 -- _CN_26619335_110000_CN_178234890_110000/LConn3 -- L_26619335/LConn3 -- bus158/LConn1
  T_167455825__/LConn1 -- _CN_35281467_110000_CN_167455825_110000/RConn1
  T_167455825__/LConn2 -- _CN_35281467_110000_CN_167455825_110000/RConn2
  _CN_35281467_110000_CN_167455825_110000/RConn3 -- T_167455825__/LConn3 -- bus159/LConn1
  T_348251886_110000_/LConn1 -- _CN_35281467_110000_CN_348251886_110000/RConn1
  T_348251886_110000_/LConn2 -- _CN_35281467_110000_CN_348251886_110000/RConn2
  _CN_35281467_110000_CN_348251886_110000/RConn3 -- T_348251886_110000_/LConn3 -- bus160/LConn1
  _CN_35281467_110000_CN_178639425_110000/RConn1 -- T_178639425_110000_/LConn1 -- _CN_178639425_110000_CN_46201634_110000/LConn1 -- _CN_178639425_110000_CN_178694062_110000/LConn1
  _CN_35281467_110000_CN_178639425_110000/RConn2 -- T_178639425_110000_/LConn2 -- _CN_178639425_110000_CN_46201634_110000/LConn2 -- _CN_178639425_110000_CN_178694062_110000/LConn2
  _CN_35281467_110000_CN_178639425_110000/RConn3 -- T_178639425_110000_/LConn3 -- _CN_178639425_110000_CN_46201634_110000/LConn3 -- _CN_178639425_110000_CN_178694062_110000/LConn3 -- bus161/LConn1
  T_46201634_110000_/LConn1 -- _CN_178639425_110000_CN_46201634_110000/RConn1
  T_46201634_110000_/LConn2 -- _CN_178639425_110000_CN_46201634_110000/RConn2
  _CN_178639425_110000_CN_46201634_110000/RConn3 -- T_46201634_110000_/LConn3 -- bus162/LConn1
  T_178694062__/LConn1 -- _CN_178639425_110000_CN_178694062_110000/RConn1
  T_178694062__/LConn2 -- _CN_178639425_110000_CN_178694062_110000/RConn2
  _CN_178639425_110000_CN_178694062_110000/RConn3 -- T_178694062__/LConn3 -- bus163/LConn1
  _CN_28258887_110000_CN_27674611_110000/LConn1 -- T_28258887__/LConn1 -- _CN_28258887_110000_CN_28484367_110000/LConn1 -- _CN_28258887_110000_CN_236712763_110000/LConn1
  _CN_28258887_110000_CN_27674611_110000/LConn2 -- T_28258887__/LConn2 -- _CN_28258887_110000_CN_28484367_110000/LConn2 -- _CN_28258887_110000_CN_236712763_110000/LConn2
  _CN_28258887_110000_CN_27674611_110000/LConn3 -- T_28258887__/LConn3 -- _CN_28258887_110000_CN_28484367_110000/LConn3 -- _CN_28258887_110000_CN_236712763_110000/LConn3 -- bus164/LConn1
  _CN_28258887_110000_CN_27674611_110000/RConn1 -- T_27674611_400000;110000_/RConn1 -- L_27674611/LConn1
  _CN_28258887_110000_CN_27674611_110000/RConn2 -- T_27674611_400000;110000_/RConn2 -- L_27674611/LConn2
  _CN_28258887_110000_CN_27674611_110000/RConn3 -- T_27674611_400000;110000_/RConn3 -- L_27674611/LConn3 -- bus165/LConn1
  T_28484367__/LConn1 -- _CN_28258887_110000_CN_28484367_110000/RConn1
  T_28484367__/LConn2 -- _CN_28258887_110000_CN_28484367_110000/RConn2
  _CN_28258887_110000_CN_28484367_110000/RConn3 -- T_28484367__/LConn3 -- bus166/LConn1
  G_236712763_/RConn1 -- _CN_28258887_110000_CN_236712763_110000/RConn1
  G_236712763_/RConn2 -- _CN_28258887_110000_CN_236712763_110000/RConn2
  _CN_28258887_110000_CN_236712763_110000/RConn3 -- G_236712763_/RConn3 -- bus167/LConn1
  _CN_142035550_110000_CN_98561229_110000/RConn1 -- T_98561229_400000;110000_/RConn1 -- _CN_98561229_110000_CN_167862173_110000/LConn1 -- L_98561229/LConn1
  _CN_142035550_110000_CN_98561229_110000/RConn2 -- T_98561229_400000;110000_/RConn2 -- _CN_98561229_110000_CN_167862173_110000/LConn2 -- L_98561229/LConn2
  _CN_142035550_110000_CN_98561229_110000/RConn3 -- T_98561229_400000;110000_/RConn3 -- _CN_98561229_110000_CN_167862173_110000/LConn3 -- L_98561229/LConn3 -- bus168/LConn1
  _CN_88283757_110000_CN_35263666_110000/LConn1 -- T_88283757_110000_/LConn1 -- _CN_88283757_110000_CN_149965739_110000/LConn1 -- _CN_88283757_110000_CN_371246420_110000/LConn1
  _CN_88283757_110000_CN_35263666_110000/LConn2 -- T_88283757_110000_/LConn2 -- _CN_88283757_110000_CN_149965739_110000/LConn2 -- _CN_88283757_110000_CN_371246420_110000/LConn2
  _CN_88283757_110000_CN_35263666_110000/LConn3 -- T_88283757_110000_/LConn3 -- _CN_88283757_110000_CN_149965739_110000/LConn3 -- _CN_88283757_110000_CN_371246420_110000/LConn3 -- bus169/LConn1
  T_35263666_110000_/LConn1 -- _CN_88283757_110000_CN_35263666_110000/RConn1
  T_35263666_110000_/LConn2 -- _CN_88283757_110000_CN_35263666_110000/RConn2
  _CN_88283757_110000_CN_35263666_110000/RConn3 -- T_35263666_110000_/LConn3 -- bus170/LConn1
  _CN_88283757_110000_CN_149965739_110000/RConn1 -- T_149965739_400000;110000_/RConn1 -- L_149965739/LConn1
  _CN_88283757_110000_CN_149965739_110000/RConn2 -- T_149965739_400000;110000_/RConn2 -- L_149965739/LConn2
  _CN_88283757_110000_CN_149965739_110000/RConn3 -- T_149965739_400000;110000_/RConn3 -- L_149965739/LConn3 -- bus171/LConn1
  T_371246420_110000_/LConn1 -- _CN_88283757_110000_CN_371246420_110000/RConn1
  T_371246420_110000_/LConn2 -- _CN_88283757_110000_CN_371246420_110000/RConn2
  _CN_88283757_110000_CN_371246420_110000/RConn3 -- T_371246420_110000_/LConn3 -- bus172/LConn1
  Tuovila_Vaskiluoto_CN_93624966_110000_CN_150209972_110000/RConn1 -- T_93624966_110000_/LConn1 -- Tuovila_Vaskiluoto_CN_93624966_110000_CN_57845262_110000/RConn1
  Tuovila_Vaskiluoto_CN_93624966_110000_CN_150209972_110000/RConn2 -- T_93624966_110000_/LConn2 -- Tuovila_Vaskiluoto_CN_93624966_110000_CN_57845262_110000/RConn2
  Tuovila_Vaskiluoto_CN_93624966_110000_CN_150209972_110000/RConn3 -- T_93624966_110000_/LConn3 -- Tuovila_Vaskiluoto_CN_93624966_110000_CN_57845262_110000/RConn3 -- bus173/LConn1
  T_169018002__/LConn1 -- _CN_169018002_110000_CN_59014204_110000/RConn1
  T_169018002__/LConn2 -- _CN_169018002_110000_CN_59014204_110000/RConn2
  _CN_169018002_110000_CN_59014204_110000/RConn3 -- T_169018002__/LConn3 -- bus174/LConn1
  _CN_168049346_110000_CN_123462491_110000/RConn1 -- T_123462491_400000;110000_Empower/RConn1 -- L_123462491/LConn1
  _CN_168049346_110000_CN_123462491_110000/RConn2 -- T_123462491_400000;110000_Empower/RConn2 -- L_123462491/LConn2
  _CN_168049346_110000_CN_123462491_110000/RConn3 -- T_123462491_400000;110000_Empower/RConn3 -- L_123462491/LConn3 -- bus175/LConn1
  _CN_168049346_110000_CN_167040166_110000/RConn1 -- G_167040166_/RConn1 -- _CN_159172094_110000_CN_167040166_110000/LConn1
  _CN_168049346_110000_CN_167040166_110000/RConn2 -- G_167040166_/RConn2 -- _CN_159172094_110000_CN_167040166_110000/LConn2
  _CN_168049346_110000_CN_167040166_110000/RConn3 -- G_167040166_/RConn3 -- _CN_159172094_110000_CN_167040166_110000/LConn3 -- bus176/LConn1
  _CN_220230343_110000_CN_205715364_110000/RConn1 -- T_220230343_110000_/LConn1 -- _CN_220230343_110000_CN_208979069_110000/RConn1 -- _CN_220230343_110000_CN_220230350_110000/LConn1
  _CN_220230343_110000_CN_205715364_110000/RConn2 -- T_220230343_110000_/LConn2 -- _CN_220230343_110000_CN_208979069_110000/RConn2 -- _CN_220230343_110000_CN_220230350_110000/LConn2
  _CN_220230343_110000_CN_205715364_110000/RConn3 -- T_220230343_110000_/LConn3 -- _CN_220230343_110000_CN_208979069_110000/RConn3 -- _CN_220230343_110000_CN_220230350_110000/LConn3 -- bus177/LConn1
  T_220230350_110000_/LConn1 -- _CN_220230343_110000_CN_220230350_110000/RConn1
  T_220230350_110000_/LConn2 -- _CN_220230343_110000_CN_220230350_110000/RConn2
  _CN_220230343_110000_CN_220230350_110000/RConn3 -- T_220230350_110000_/LConn3 -- bus178/LConn1
  T_36977363__/LConn1 -- _CN_36977363_110000_CN_6268760_110000/RConn1
  T_36977363__/LConn2 -- _CN_36977363_110000_CN_6268760_110000/RConn2
  _CN_36977363_110000_CN_6268760_110000/RConn3 -- T_36977363__/LConn3 -- bus179/LConn1
  _CN_130331348_110000_CN_150204241_110000/RConn1 -- T_150204241_110000_/LConn1 -- _CN_252609822_110000_CN_150204241_110000/LConn1
  _CN_130331348_110000_CN_150204241_110000/RConn2 -- T_150204241_110000_/LConn2 -- _CN_252609822_110000_CN_150204241_110000/LConn2
  _CN_130331348_110000_CN_150204241_110000/RConn3 -- T_150204241_110000_/LConn3 -- _CN_252609822_110000_CN_150204241_110000/LConn3 -- bus180/LConn1
  T_94091993_110000_/LConn1 -- _CN_94091993_110000_CN_93582884_110000/LConn1
  T_94091993_110000_/LConn2 -- _CN_94091993_110000_CN_93582884_110000/LConn2
  _CN_94091993_110000_CN_93582884_110000/LConn3 -- T_94091993_110000_/LConn3 -- bus181/LConn1
  T_93582884_110000_/LConn1 -- _CN_94091993_110000_CN_93582884_110000/RConn1
  T_93582884_110000_/LConn2 -- _CN_94091993_110000_CN_93582884_110000/RConn2
  _CN_94091993_110000_CN_93582884_110000/RConn3 -- T_93582884_110000_/LConn3 -- bus182/LConn1
  T_158104293_110000_/LConn1 -- _CN_158104293_110000_CN_98736918_110000/RConn1
  T_158104293_110000_/LConn2 -- _CN_158104293_110000_CN_98736918_110000/RConn2
  _CN_158104293_110000_CN_98736918_110000/RConn3 -- T_158104293_110000_/LConn3 -- bus183/LConn1
  T_319750899_110000;20000_Fortum/LConn1 -- _CN_319750899_110000_CN_95392702_110000/LConn1
  T_319750899_110000;20000_Fortum/LConn2 -- _CN_319750899_110000_CN_95392702_110000/LConn2
  _CN_319750899_110000_CN_95392702_110000/LConn3 -- T_319750899_110000;20000_Fortum/LConn3 -- bus184/LConn1
  _CN_319750899_110000_CN_95392702_110000/RConn1 -- T_95392702_400000;110000_400kV_Salo/RConn1 -- L_95392702/LConn1
  _CN_319750899_110000_CN_95392702_110000/RConn2 -- T_95392702_400000;110000_400kV_Salo/RConn2 -- L_95392702/LConn2
  _CN_319750899_110000_CN_95392702_110000/RConn3 -- T_95392702_400000;110000_400kV_Salo/RConn3 -- L_95392702/LConn3 -- bus185/LConn1
  _CN_348349188_110000_CN_348349190_110000/LConn1 -- T_348349188__/LConn1 -- _CN_348349188_110000_CN_40101584_110000/RConn1
  _CN_348349188_110000_CN_348349190_110000/LConn2 -- T_348349188__/LConn2 -- _CN_348349188_110000_CN_40101584_110000/RConn2
  _CN_348349188_110000_CN_348349190_110000/LConn3 -- T_348349188__/LConn3 -- _CN_348349188_110000_CN_40101584_110000/RConn3 -- bus186/LConn1
  T_348349190_110000_/LConn1 -- _CN_348349188_110000_CN_348349190_110000/RConn1
  T_348349190_110000_/LConn2 -- _CN_348349188_110000_CN_348349190_110000/RConn2
  _CN_348349188_110000_CN_348349190_110000/RConn3 -- T_348349190_110000_/LConn3 -- bus187/LConn1
  _CN_153187093_110000_CN_159935727_110000/LConn1 -- T_153187093_110000_/LConn1 -- _CN_153187093_110000_CN_128463750_110000/RConn1
  _CN_153187093_110000_CN_159935727_110000/LConn2 -- T_153187093_110000_/LConn2 -- _CN_153187093_110000_CN_128463750_110000/RConn2
  _CN_153187093_110000_CN_159935727_110000/LConn3 -- T_153187093_110000_/LConn3 -- _CN_153187093_110000_CN_128463750_110000/RConn3 -- bus188/LConn1
  T_159935727__/LConn1 -- _CN_153187093_110000_CN_159935727_110000/RConn1
  T_159935727__/LConn2 -- _CN_153187093_110000_CN_159935727_110000/RConn2
  _CN_153187093_110000_CN_159935727_110000/RConn3 -- T_159935727__/LConn3 -- bus189/LConn1
  _CN_98736918_110000_CN_158031219_110000/RConn1 -- T_158031219_110000_/LConn1 -- _CN_158219552_110000_CN_158031219_110000/LConn1
  _CN_98736918_110000_CN_158031219_110000/RConn2 -- T_158031219_110000_/LConn2 -- _CN_158219552_110000_CN_158031219_110000/LConn2
  _CN_98736918_110000_CN_158031219_110000/RConn3 -- T_158031219_110000_/LConn3 -- _CN_158219552_110000_CN_158031219_110000/LConn3 -- bus190/LConn1
  _CN_26391332_110000_CN_25593756_110000/RConn1 -- T_26391332__Pitajanmaki/LConn1 -- _CN_26391332_110000_CN_26367884_110000/LConn1
  _CN_26391332_110000_CN_25593756_110000/RConn2 -- T_26391332__Pitajanmaki/LConn2 -- _CN_26391332_110000_CN_26367884_110000/LConn2
  _CN_26391332_110000_CN_25593756_110000/RConn3 -- T_26391332__Pitajanmaki/LConn3 -- _CN_26391332_110000_CN_26367884_110000/LConn3 -- bus191/LConn1
